simulink model "x35BusNetworkElectricityTransmissionModel"  (R2023b)
settings: Solver=VariableStepAuto  StartTime=0.0  StopTime=0.8  RelTol=1e-3
model workspace (MAT data in the model file):
  Compensation_Ki = 30
  Compensation_Kp = 3
  DC_Ki = 400
  DC_Kp = 8
  F = 0.01
  Flux_min = 0.5
  Grid_Freq_PWM = 2700
  Grid_Ireg_Ki = 5
  Grid_Ireg_Kp = 0.83
  Grid_Ireg_lim = 1.1
  Grid_Modindex_Upper = 1.1
  Grid_conv_Imax = 0.8
  H = 0.685
  Idref_max = 0.9
  Iqref_Tc = 0.3
  Ki_Var = 0.05
  Ki_Vreg = 20
  Ksh = 1.1
  L_pu = 0.3
  Llr = 0.16
  Lls = 0.18
  Lm = 2.9
  Nb_wt = 6
  P_mech = 1080000
  Pitch_Ki = 0
  Pitch_Kp = 150
  Pitch_Max = 27
  Pitch_Tc = 0.01
  Pitch_rate = 10
  Q_Filt = 50
  R_pu = 0.003
  Rotor_Freq_PWM = 1620
  Rotor_Ireg_Ki = 8
  Rotor_Ireg_Kp = 0.6
  Rotor_Ireg_lim = 0.1
  Rotor_Modindex_Upper = 2
  Rr = 0.016
  Rs = 0.023
  T_set = 0.0001
  Tp = 5e-05
  Ts = 5e-06
  Var_C_Filt = 720000
  Var_reg_max = 1.1
  Var_reg_min = 0.9
  WT_Coeff = [0.645 116 0.4 5 21 0.00912 0.08 0.035]
  WT_H = 4.32
  WT_IGBTRon = 5.931
  WT_Param = [91.204 10143]
  Wind_Freq_Filt = 10000
  Wind_Freq_nom = 60
  Wind_P_nom = 1200000
  Wind_Rotor_V_nom = 1950
  Wind_V_nom = 500
  Zeta_Filt = 0.707106781187
  init = [-0.2 0 0 0 0 0 0 0]
  p = 3
  torque0 = 0.83
  v_Ki = 0.1
  v_Kp = 3.6
  v_Max = 1.2
  v_Min = 0.7
  v_T = 5
  vreg_max = 1
  wind_VDC_nom = 1150
  wt0 = 1.2
undefined symbols (not defined in the file): D1, D11, Delta, DiscIntNeverNeededParam, Ion, Lithium, P, Q
libraries: powerlib_extras x144, spsSeriesRLCBranchLib x67, spsLoadFlowBusLib x43, spsThreePhaseTransformerTwoWindingsLib x32, spsThreePhaseSeriesRLCLoadLib x31, spsThreePhaseVIMeasurementLib x26, simulink_extras x26, spsDistributedParametersLineLib x22, spsGenericPowerSystemStabilizerLib x20, spsSynchronousMachinepuStandardLib x10, spsExcitationSystemLib x10, spsHydraulicTurbineandGovernorLib x10
(part 5 of 16)

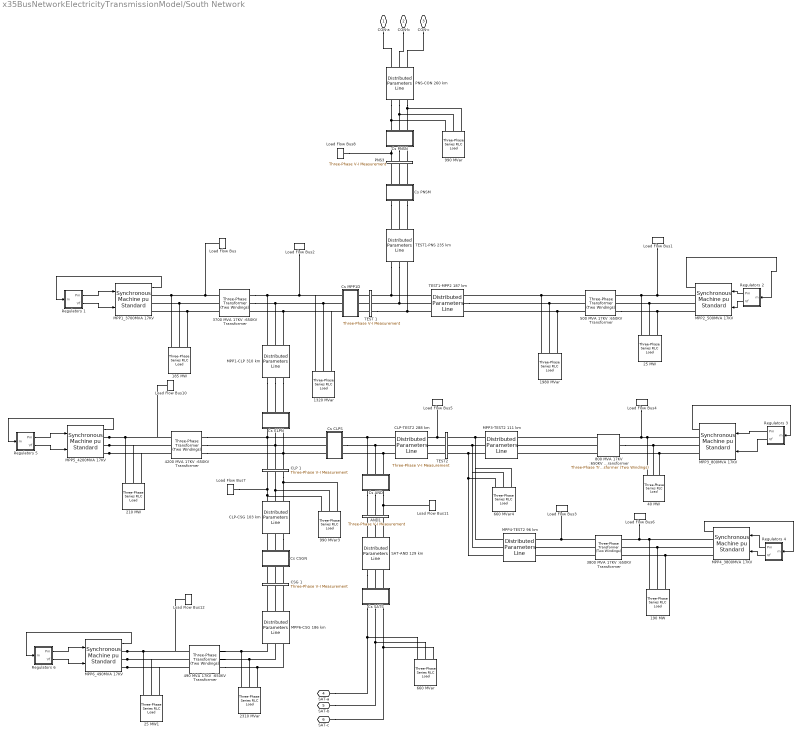
== system x35BusNetworkElectricityTransmissionModel/South Network ==
  " SAT-AND 129 km" : spsDistributedParametersLineLib/Distributed Parameters Line  Phases=3  Length=129  Frequency=60  Resistance=[0.01273 0.3864]/6  Inductance="[0.9337e-3  4.1264e-3]/6"  Capacitance=[12.74e-9 7.751e-9]*6  x1=[-0.00078 1.73015070651852e-08 -160788.800409401 -239334.964150814;-0.00072 1.8256737808598e-08 -155334.496074464 -242910.417917869;-0.00066 1.92026280676021e-08 -149800.719741084 -246361.594226648;-0.0006 2.01386939072632e-08 -144190.302591486 -249686.727391582;-0.00054 2.10644564190009e-08 -138506.115018751 -252884.116213103;-0.00048 2.19794419656084e-08 -132751.065158274 -255952.124848007;-0.00042 2.28831824235728e-08 -126928.097399904 -258889.183646388;-0.00036 2.37752154225767e-08 -121040.190881543 -261693.789954693;-0.0003 2.4655084582055e-08 -115090.357964961 -264364.508884513;-0.00024 2.55223397446875e-08 -109081.642694619 -266899.974046692;-0.00018 2.6376537206708e-08 -103017.119240278 -269298.888250405;-0.00012 2.72172399449112e-08 -96899.8903241954 -271560.024166817;-6e-05 2.80440178402418e-08 -90733.0856337191 -273682.224957013]  x2=[-0.00078 5.22592266110193e-08 -88973.713875581 -231973.83539445;-0.00072 5.48882545652481e-08 -83704.2752060405 -233926.888762085;-0.00066 5.7489200674223e-08 -78392.0118826275 -235760.260810956;-0.0006 6.00607342458547e-08 -73039.6417574174 -237473.013554048;-0.00054 6.26015396360514e-08 -67649.9032018668 -239064.27071541;-0.00048 6.51103169218269e-08 -62225.5537058117 -240533.218178473;-0.00042 6.75857825663648e-08 -56769.3684666847 -241879.104402573;-0.00036 7.00266700757002e-08 -51284.1389696728 -243101.240807449;-0.0003 7.24317306466807e-08 -45772.671559542 -244199.002125534;-0.00024 7.47997338058778e-08 -40237.7860048597 -245171.826721852;-0.00018 7.71294680391197e-08 -34682.3140553485 -246019.216881365;-0.00012 7.94197414113241e-08 -29109.0979931111 -246740.739063609;-6e-05 8.16693821763144e-08 -23520.9891784661 -247336.024124503]  x3=[-0.00078 -1.72880421705233e-09 -2677.59154686044 -14439.5075300877;-0.00072 -1.68724420508278e-09 -2350.32071608935 -14496.375500878;-0.00066 -1.64482096780123e-09 -2021.84741781098 -14545.8268580998;-0.0006 -1.60155620971975e-09 -1692.33970503421 -14587.8363015251;-0.00054 -1.55747206588802e-09 -1361.96615999351 -14622.3823383462;-0.00048 -1.51259109056861e-09 -1030.89580789911 -14649.4472941725;-0.00042 -1.4669362456978e-09 -699.298030460621 -14669.0173220725;-0.00036 -1.42053088913782e-09 -367.34247922821 -14681.0824096582;-0.0003 -1.37339876272656e-09 -35.1989887957174 -14685.6363842078;-0.00024 -1.32556398013081e-09 296.962510089846 -14682.676915824;-0.00018 -1.27705101450921e-09 628.972077468011 -14672.2055186254;-0.00012 -1.2278846859914e-09 960.659851109276 -14654.2275499722;-6e-05 -1.17809014897953e-09 1291.85613341976 -14628.7522077255]  x4=[-0.00078 2.10158311278446e-09 -3708.19041372056 4505.23785529734;-0.00072 2.08978742581233e-09 -3809.13872188143 4420.21514552939;-0.00066 2.07692256497832e-09 -3908.1382042874 4332.93097201679;-0.0006 2.06299511218296e-09 -4005.13821097396 4243.42999095556;-0.00054 2.04801219296843e-09 -4100.08911494535 4151.75799270137;-0.00048 2.03198147287307e-09 -4192.94233756459 4057.96187834246;-0.00042 2.01491115350949e-09 -4283.65037340727 3962.08963570407;-0.00036 1.99680996836849e-09 -4372.16681456616 3864.19031479706;-0.0003 1.97768717835087e-09 -4458.44637439435 3764.31400272297;-0.00024 1.95755256702935e-09 -4542.4449106748 3662.51179804856;-0.00018 1.93641643564312e-09 -4624.11944820421 3558.83578466283;-0.00012 1.91428959782756e-09 -4703.42820078001 3453.33900512995;-6e-05 1.89118337408174e-09 -4780.33059257894 3346.07543355167]  x5=0.000729548621424508  V1=[2.188e-18 3.182e-07 3.182e-07;377 377 377;0.6306 1.295 -0.2758]  V2=[1.209e-19 1.011e-07 1.011e-07;377 377 377;-2.255 -1.798 2.915]  I1=[1.016e-20 9.164e-09 9.164e-09;377 377 377;2.19 2.786 1.215]  I2=[1.089e-20 9.22e-09 9.22e-09;377 377 377;-0.7019 -0.2685 -1.839]  nHarmo=1  Measurements=None  Decoupling=off  VsMag0=0  VrMag0=0  VsAngle0=0  VrAngle0=0  IsMag0=0  IrMag0=0  IsAngle0=0  IrAngle0=0
      settings: LibrarySourceBlock=sps_lib/Power Grid Elements/Distributed Parameters Line
  1320 MVar : spsThreePhaseSeriesRLCLoadLib/Three-Phase Series RLC Load  LConnTagsString=A|B|C  Configuration=Y (grounded)  NominalVoltage=650e3  Vabc=[1e3 1e3 1e3]  Vabcp=[1e3 1e3 1e3]  NominalFrequency=60  UnbalancedPower=off  ActivePower=4400e3  InductivePower=1320e6  CapacitivePower=0  Pabc=[10e3 9e3 11e3]  QLabc=[100 90 110]  QCabc=[100 90 110]  Pabcp=[10e3 9e3 11e3]  QLabcp=[100 90 110]  QCabcp=[100 90 110]  Measurements=None  LoadType=constant Z
  185 MW : spsThreePhaseSeriesRLCLoadLib/Three-Phase Series RLC Load  LConnTagsString=A|B|C  Configuration=Y (grounded)  NominalVoltage=17e3  Vabc=[1e3 1e3 1e3]  Vabcp=[1e3 1e3 1e3]  NominalFrequency=60  UnbalancedPower=off  ActivePower=185e6  InductivePower=0  CapacitivePower=0  Pabc=[10e3 9e3 11e3]  QLabc=[100 90 110]  QCabc=[100 90 110]  Pabcp=[10e3 9e3 11e3]  QLabcp=[100 90 110]  QCabcp=[100 90 110]  Measurements=None  LoadType=constant Z
  190 MW : spsThreePhaseSeriesRLCLoadLib/Three-Phase Series RLC Load  LConnTagsString=A|B|C  Configuration=Y (grounded)  NominalVoltage=17e3  Vabc=[1e3 1e3 1e3]  Vabcp=[1e3 1e3 1e3]  NominalFrequency=60  UnbalancedPower=off  ActivePower=190e6  InductivePower=0  CapacitivePower=0  Pabc=[10e3 9e3 11e3]  QLabc=[100 90 110]  QCabc=[100 90 110]  Pabcp=[10e3 9e3 11e3]  QLabcp=[100 90 110]  QCabcp=[100 90 110]  Measurements=None  LoadType=constant Z
  1980 MVar : spsThreePhaseSeriesRLCLoadLib/Three-Phase Series RLC Load  LConnTagsString=A|B|C  Configuration=Y (grounded)  NominalVoltage=650e3  Vabc=[1e3 1e3 1e3]  Vabcp=[1e3 1e3 1e3]  NominalFrequency=60  UnbalancedPower=off  ActivePower=4400e3  InductivePower=1320e6  CapacitivePower=0  Pabc=[10e3 9e3 11e3]  QLabc=[100 90 110]  QCabc=[100 90 110]  Pabcp=[10e3 9e3 11e3]  QLabcp=[100 90 110]  QCabcp=[100 90 110]  Measurements=None  LoadType=constant Z
  210 MW : spsThreePhaseSeriesRLCLoadLib/Three-Phase Series RLC Load  LConnTagsString=A|B|C  Configuration=Y (grounded)  NominalVoltage=17e3  Vabc=[1e3 1e3 1e3]  Vabcp=[1e3 1e3 1e3]  NominalFrequency=60  UnbalancedPower=off  ActivePower=210e6  InductivePower=0  CapacitivePower=0  Pabc=[10e3 9e3 11e3]  QLabc=[100 90 110]  QCabc=[100 90 110]  Pabcp=[10e3 9e3 11e3]  QLabcp=[100 90 110]  QCabcp=[100 90 110]  Measurements=None  LoadType=constant Z
  2310 MVar : spsThreePhaseSeriesRLCLoadLib/Three-Phase Series RLC Load  LConnTagsString=A|B|C  Configuration=Y (grounded)  NominalVoltage=650e3  Vabc=[1e3 1e3 1e3]  Vabcp=[1e3 1e3 1e3]  NominalFrequency=60  UnbalancedPower=off  ActivePower=7700e3  InductivePower=2310e6  CapacitivePower=0  Pabc=[10e3 9e3 11e3]  QLabc=[100 90 110]  QCabc=[100 90 110]  Pabcp=[10e3 9e3 11e3]  QLabcp=[100 90 110]  QCabcp=[100 90 110]  Measurements=None  LoadType=constant Z
  25 MW : spsThreePhaseSeriesRLCLoadLib/Three-Phase Series RLC Load  LConnTagsString=A|B|C  Configuration=Y (grounded)  NominalVoltage=17e3  Vabc=[1e3 1e3 1e3]  Vabcp=[1e3 1e3 1e3]  NominalFrequency=60  UnbalancedPower=off  ActivePower=25e6  InductivePower=0  CapacitivePower=0  Pabc=[10e3 9e3 11e3]  QLabc=[100 90 110]  QCabc=[100 90 110]  Pabcp=[10e3 9e3 11e3]  QLabcp=[100 90 110]  QCabcp=[100 90 110]  Measurements=None  LoadType=constant Z
  25 MW1 : spsThreePhaseSeriesRLCLoadLib/Three-Phase Series RLC Load  LConnTagsString=A|B|C  Configuration=Y (grounded)  NominalVoltage=17e3  Vabc=[1e3 1e3 1e3]  Vabcp=[1e3 1e3 1e3]  NominalFrequency=60  UnbalancedPower=off  ActivePower=25e6  InductivePower=0  CapacitivePower=0  Pabc=[10e3 9e3 11e3]  QLabc=[100 90 110]  QCabc=[100 90 110]  Pabcp=[10e3 9e3 11e3]  QLabcp=[100 90 110]  QCabcp=[100 90 110]  Measurements=None  LoadType=constant Z
  "3700 MVA 17KV :650KV Transformer " : spsThreePhaseTransformerTwoWindingsLib/Three-Phase Transformer (Two Windings)  Winding1Connection=Delta (D1)  Winding2Connection=Yg  CoreType=Three single-phase transformers  SetSaturation=off  Hysteresis=off  DataFile='hysteresis'  SetInitialFlux=off  Measurements=None  UNITS=pu  NominalPower=[ 3700e6 , 60 ]  Winding1=[ 17e3 , 0.002 , 0.08 ]  Winding2=[ 650e3 , 0.002 , 0.08 ]  Rm=500  Lm=500  L0=0.5  Saturation=[ 0,0 ; 0.0024,1.2 ; 1.0,1.52 ]  InitialFluxes=[ 0.8 , -0.8 , 0.7 ]  BreakLoop=off  DiscreteSolver=Trapezoidal iterative  DataType=off  TransfoNumber=1
  3800 MVA 17KV :650KV Transformer : spsThreePhaseTransformerTwoWindingsLib/Three-Phase Transformer (Two Windings)  Winding1Connection=Yg  Winding2Connection=Delta (D1)  CoreType=Three single-phase transformers  SetSaturation=off  Hysteresis=off  DataFile='hysteresis'  SetInitialFlux=off  Measurements=None  UNITS=pu  NominalPower=[ 3800e6 , 60 ]  Winding1=[ 650e3 , 0.002 , 0.08 ]  Winding2=[ 17e3 , 0.002 , 0.08 ]  Rm=500  Lm=500  L0=0.5  Saturation=[ 0,0 ; 0.0024,1.2 ; 1.0,1.52 ]  InitialFluxes=[ 0.8 , -0.8 , 0.7 ]  BreakLoop=off  DiscreteSolver=Trapezoidal iterative  DataType=off  TransfoNumber=1
  40 MW : spsThreePhaseSeriesRLCLoadLib/Three-Phase Series RLC Load  LConnTagsString=A|B|C  Configuration=Y (grounded)  NominalVoltage=17e3  Vabc=[1e3 1e3 1e3]  Vabcp=[1e3 1e3 1e3]  NominalFrequency=60  UnbalancedPower=off  ActivePower=40e6  InductivePower=0  CapacitivePower=0  Pabc=[10e3 9e3 11e3]  QLabc=[100 90 110]  QCabc=[100 90 110]  Pabcp=[10e3 9e3 11e3]  QLabcp=[100 90 110]  QCabcp=[100 90 110]  Measurements=None  LoadType=constant Z
  4200 MVA 17KV :650KV Transformer : spsThreePhaseTransformerTwoWindingsLib/Three-Phase Transformer (Two Windings)  Winding1Connection=Delta (D1)  Winding2Connection=Yg  CoreType=Three single-phase transformers  SetSaturation=off  Hysteresis=off  DataFile='hysteresis'  SetInitialFlux=off  Measurements=None  UNITS=pu  NominalPower=[ 4200e6 , 60 ]  Winding1=[ 17e3 , 0.002 , 0.08 ]  Winding2=[ 650e3 , 0.002 , 0.08 ]  Rm=500  Lm=500  L0=0.5  Saturation=[ 0,0 ; 0.0024,1.2 ; 1.0,1.52 ]  InitialFluxes=[ 0.8 , -0.8 , 0.7 ]  BreakLoop=off  DiscreteSolver=Trapezoidal iterative  DataType=off  TransfoNumber=1
  490 MVA 17KV :650KV Transformer : spsThreePhaseTransformerTwoWindingsLib/Three-Phase Transformer (Two Windings)  Winding1Connection=Delta (D1)  Winding2Connection=Yg  CoreType=Three single-phase transformers  SetSaturation=off  Hysteresis=off  DataFile='hysteresis'  SetInitialFlux=off  Measurements=None  UNITS=pu  NominalPower=[ 490e6 , 60 ]  Winding1=[ 17e3 , 0.002 , 0.08 ]  Winding2=[ 650e3 , 0.002 , 0.08 ]  Rm=500  Lm=500  L0=0.5  Saturation=[ 0,0 ; 0.0024,1.2 ; 1.0,1.52 ]  InitialFluxes=[ 0.8 , -0.8 , 0.7 ]  BreakLoop=off  DiscreteSolver=Trapezoidal iterative  DataType=off  TransfoNumber=1
  "500 MVA 17KV :650KV Transformer " : spsThreePhaseTransformerTwoWindingsLib/Three-Phase Transformer (Two Windings)  Winding1Connection=Yg  Winding2Connection=Delta (D1)  CoreType=Three single-phase transformers  SetSaturation=off  Hysteresis=off  DataFile='hysteresis'  SetInitialFlux=off  Measurements=None  UNITS=pu  NominalPower=[ 500e6 , 60 ]  Winding1=[650e3 , 0.002 , 0.08 ]  Winding2=[17e3 , 0.002 , 0.08 ]  Rm=500  Lm=500  L0=0.5  Saturation=[ 0,0 ; 0.0024,1.2 ; 1.0,1.52 ]  InitialFluxes=[ 0.8 , -0.8 , 0.7 ]  BreakLoop=off  DiscreteSolver=Trapezoidal iterative  DataType=off  TransfoNumber=1
  660 MVar : spsThreePhaseSeriesRLCLoadLib/Three-Phase Series RLC Load  LConnTagsString=A|B|C  Configuration=Y (grounded)  NominalVoltage=650e3  Vabc=[1e3 1e3 1e3]  Vabcp=[1e3 1e3 1e3]  NominalFrequency=60  UnbalancedPower=off  ActivePower=2200e3  InductivePower=660e6  CapacitivePower=0  Pabc=[10e3 9e3 11e3]  QLabc=[100 90 110]  QCabc=[100 90 110]  Pabcp=[10e3 9e3 11e3]  QLabcp=[100 90 110]  QCabcp=[100 90 110]  Measurements=None  LoadType=constant Z
  660 MVar4 : spsThreePhaseSeriesRLCLoadLib/Three-Phase Series RLC Load  LConnTagsString=A|B|C  Configuration=Y (grounded)  NominalVoltage=650e3  Vabc=[1e3 1e3 1e3]  Vabcp=[1e3 1e3 1e3]  NominalFrequency=60  UnbalancedPower=off  ActivePower=2200e3  InductivePower=660e6  CapacitivePower=0  Pabc=[10e3 9e3 11e3]  QLabc=[100 90 110]  QCabc=[100 90 110]  Pabcp=[10e3 9e3 11e3]  QLabcp=[100 90 110]  QCabcp=[100 90 110]  Measurements=None  LoadType=constant Z
  800 MVA 17KV :650KV Transformer : spsThreePhaseTransformerTwoWindingsLib/Three-Phase Transformer (Two Windings)  Winding1Connection=Yg  Winding2Connection=Delta (D1)  CoreType=Three single-phase transformers  SetSaturation=off  Hysteresis=off  DataFile='hysteresis'  SetInitialFlux=off  Measurements=None  UNITS=pu  NominalPower=[ 800e6 , 60 ]  Winding1=[650e3 , 0.002 , 0.08 ]  Winding2=[ 17e3 , 0.002 , 0.08 ]  Rm=500  Lm=500  L0=0.5  Saturation=[ 0,0 ; 0.0024,1.2 ; 1.0,1.52 ]  InitialFluxes=[ 0.8 , -0.8 , 0.7 ]  BreakLoop=off  DiscreteSolver=Trapezoidal iterative  DataType=off  TransfoNumber=1
  990 MVar : spsThreePhaseSeriesRLCLoadLib/Three-Phase Series RLC Load  LConnTagsString=A|B|C  Configuration=Y (grounded)  NominalVoltage=650e3  Vabc=[1e3 1e3 1e3]  Vabcp=[1e3 1e3 1e3]  NominalFrequency=60  UnbalancedPower=off  ActivePower=2200e3  InductivePower=660e6  CapacitivePower=0  Pabc=[10e3 9e3 11e3]  QLabc=[100 90 110]  QCabc=[100 90 110]  Pabcp=[10e3 9e3 11e3]  QLabcp=[100 90 110]  QCabcp=[100 90 110]  Measurements=None  LoadType=constant Z
  990 MVar3 : spsThreePhaseSeriesRLCLoadLib/Three-Phase Series RLC Load  LConnTagsString=A|B|C  Configuration=Y (grounded)  NominalVoltage=650e3  Vabc=[1e3 1e3 1e3]  Vabcp=[1e3 1e3 1e3]  NominalFrequency=60  UnbalancedPower=off  ActivePower=3300e3  InductivePower=990e6  CapacitivePower=0  Pabc=[10e3 9e3 11e3]  QLabc=[100 90 110]  QCabc=[100 90 110]  Pabcp=[10e3 9e3 11e3]  QLabcp=[100 90 110]  QCabcp=[100 90 110]  Measurements=None  LoadType=constant Z
  AND1 : spsThreePhaseVIMeasurementLib/Three-Phase V-I Measurement  VoltageMeasurement=no  SetLabelV=off  LabelV=Vabc  Vpu=off  VpuLL=off  CurrentMeasurement=no  SetLabelI=off  LabelI=Iabc  Ipu=off  Pbase=100e6  Vbase=500e3  OutputType=Complex  PhasorSimulation=off  PSBequivalent=0
  CLP 1 : spsThreePhaseVIMeasurementLib/Three-Phase V-I Measurement  VoltageMeasurement=no  SetLabelV=off  LabelV=Vabc  Vpu=off  VpuLL=off  CurrentMeasurement=no  SetLabelI=off  LabelI=Iabc  Ipu=off  Pbase=100e6  Vbase=500e3  OutputType=Complex  PhasorSimulation=off  PSBequivalent=0
  CLP-CSG 103 km : spsDistributedParametersLineLib/Distributed Parameters Line  Phases=3  Length=103  Frequency=60  Resistance=[0.01273 0.3864]/6  Inductance="[0.9337e-3  4.1264e-3]/6"  Capacitance=[12.74e-9 7.751e-9]*6  x1=[-0.0006 3.92711037156733e-08 -150312.081292197 -256752.693722347;-0.00054 4.02003694351059e-08 -144466.512887676 -260086.735304661;-0.00048 4.1109067902718e-08 -138547.032745726 -263287.711707343;-0.00042 4.19967342115829e-08 -132556.669381769 -266353.985251718;-0.00036 4.28629142152147e-08 -126498.487576391 -269283.987175583;-0.0003 4.37071647599184e-08 -120375.586807346 -272076.218435812;-0.00024 4.45290539115154e-08 -114191.099663804 -274729.250475299;-0.00018 4.53281611763289e-08 -107948.190243666 -277241.72595383;-0.00012 4.61040777163166e-08 -101650.052534746 -279612.359442526;-6e-05 4.68564065582391e-08 -95299.908780672 -281839.938081488]  x2=[-0.0006 3.46834464690486e-08 -152766.904511302 -257465.980570063;-0.00054 3.58237170617729e-08 -146904.575209073 -260855.361892625;-0.00048 3.69456595789022e-08 -140967.086811682 -264111.28479199;-0.00042 3.80487000139136e-08 -134957.477047906 -267232.08347784;-0.00036 3.91322740309387e-08 -128878.820545144 -270216.161291901;-0.0003 4.01958272534884e-08 -122734.227256386 -273061.991524825;-0.00024 4.12388155480817e-08 -116526.840869094 -275768.118197279;-0.00018 4.22607053026349e-08 -110259.837196846 -278333.156804855;-0.00012 4.32609736994672e-08 -103936.422554521 -280755.795026404;-6e-05 4.42391089827839e-08 -97559.8321178918 -283034.793395447]  x3=[-0.0006 -8.57836265093248e-11 -3832.5749236527 -5045.22121215062;-0.00054 -7.93836822522111e-11 -3717.48388598462 -5130.61468863092;-0.00048 -7.29431238364154e-11 -3600.49091486927 -5213.38324783366;-0.00042 -6.6465246370631e-11 -3481.65586607244 -5293.48454383456;-0.00036 -5.99533640566669e-11 -3361.03953780094 -5370.87759533049;-0.0003 -5.34108084938405e-11 -3238.70363959702 -5445.52280660624;-0.00024 -4.68409269744705e-11 -3114.71076076672 -5517.38198779243;-0.00018 -4.02470807713395e-11 -2989.12433835798 -5586.41837440418;-0.00012 -3.36326434180053e-11 -2862.00862470507 -5652.59664615044;-6e-05 -2.70009989828387e-11 -2733.42865455591 -5715.88294500454]  x4=[-0.0006 5.88767514656271e-10 -3622.67392283929 -5860.74468145355;-0.00054 6.00102975589294e-10 -3489.19149359268 -5941.18214271376;-0.00048 6.11131412751377e-10 -3353.92392950511 -6018.57998540933;-0.00042 6.21847183790286e-10 -3216.94043596181 -6092.89861137379;-0.00036 6.32244806319553e-10 -3078.31109624924 -6164.09999782485;-0.0003 6.42318960723366e-10 -2938.10683569919 -6232.14771681756;-0.00024 6.52064492878184e-10 -2796.39938540202 -6297.00695388149;-0.00018 6.61476416789678e-10 -2653.26124550776 -6358.6445258325;-0.00012 6.70549917143664e-10 -2508.76564813367 -6417.02889774986;-6e-05 6.79280351769702e-10 -2362.98651989733 -6472.13019911006]  x5=0.000582507814005615  V1=[1.056e-22 6.221e-12 6.221e-12;377 377 377;0.3647 1.373 -0.1974]  V2=[1.588e-22 9.824e-12 9.824e-12;377 377 377;0.3755 1.375 -0.1957]  I1=[3.913e-25 1.044e-13 1.044e-13;377 377 377;-0.5956 0.0636 -1.507]  I2=[3.097e-25 1.021e-13 1.021e-13;377 377 377;1.525 2.624 1.053]  nHarmo=1  Measurements=None  Decoupling=off  VsMag0=0  VrMag0=0  VsAngle0=0  VrAngle0=0  IsMag0=0  IrMag0=0  IsAngle0=0  IrAngle0=0
      settings: LibrarySourceBlock=sps_lib/Power Grid Elements/Distributed Parameters Line
  CLP-TEST2 288 km : spsDistributedParametersLineLib/Distributed Parameters Line  Phases=3  Length=288  Frequency=60  Resistance=[0.01273 0.3864]/6  Inductance="[0.9337e-3  4.1264e-3]/6"  Capacitance=[12.74e-9 7.751e-9]*6  x1=[-0.00168 -5.65553918327e-09 0 0;-0.00162 -5.14288112742245e-09 0 0;-0.00156 -4.6275918785606e-09 0 0;-0.0015 -4.10993506818561e-09 0 0;-0.00144 -3.59017553908687e-09 0 0;-0.00138 -3.06857920984352e-09 0 0;-0.00132 -2.54541293877558e-09 0 0;-0.00126 -2.02094438741434e-09 0 0;-0.0012 -1.49544188356175e-09 0 0;-0.00114 -9.69174284008934e-10 0 0;-0.00108 -4.42410836984137e-10 0 0;-0.00102 8.457895559967e-11 -80544.0337060146 -208122.10077131;-0.00096 6.11525476026955e-10 -75816.2183893697 -209890.593985758;-0.0009 1.13815912872101e-09 -71049.6140944741 -211551.70329399;-0.00084 1.66421047817406e-09 -66246.6595041619 -213104.578841792;-0.00078 2.18941038679539e-09 -61409.8118987498 -214548.426149338;-0.00072 2.71349015260719e-09 -56541.5458988475 -215882.506517667;-0.00066 3.23618164671738e-09 -51644.3521992956 -217106.137406612;-0.0006 3.75721745049934e-09 -46720.7362948807 -218218.692783999;-0.00054 4.27633099240824e-09 -41773.2171984774 -219219.60344594;-0.00048 4.79325668436391e-09 -36804.326152275 -220108.357308046;-0.00042 5.30773005763066e-09 -31816.6053327474 -220884.499667418;-0.00036 5.81948789812434e-09 -26812.6065500283 -221547.633435284;-0.0003 6.32826838107758e-09 -21794.8899423582 -222097.419340155;-0.00024 6.8338112049941e-09 -16766.0226662703 -222533.576101403;-0.00018 7.33585772482384e-09 -11728.5775831858 -222855.880573169;-0.00012 7.83415108429049e-09 -6685.13194309062 -223064.167858532;-6e-05 8.32843634730394e-09 -1638.26606596631 -223158.331393866]  x2=[-0.00168 4.10808268888269e-08 0 0;-0.00162 4.02895288423073e-08 0 0;-0.00156 3.94776179283671e-08 0 0;-0.0015 3.86455095356323e-08 0 0;-0.00144 3.77936293861321e-08 0 0;-0.00138 3.6922413317492e-08 0 0;-0.00132 3.6032307059951e-08 0 0;-0.00126 3.51237660083175e-08 0 0;-0.0012 3.41972549889817e-08 0 0;-0.00114 3.32532480221008e-08 0 0;-0.00108 3.22922280790825e-08 0 0;-0.00102 3.13146868354871e-08 -161682.012206487 -227631.966150118;-0.00096 3.03211244194778e-08 -156492.170905739 -231230.614921688;-0.0009 2.93120491559456e-08 -151222.265318713 -234710.961838014;-0.00084 2.82879773064408e-08 -145874.991626483 -238071.226289303;-0.00078 2.72494328050443e-08 -140453.085593078 -241309.689102173;-0.00072 2.61969469903131e-08 -134959.321165808 -244424.693419207;-0.00066 2.51310583334377e-08 -129396.509056068 -247414.645546639;-0.0006 2.40523121627504e-08 -123767.495301323 -250278.015769713;-0.00054 2.2961260384725e-08 -118075.159809021 -253013.339135312;-0.00048 2.18584612016114e-08 -112322.414883183 -255619.216201462;-0.00042 2.07444788258492e-08 -106512.203734411 -258094.313753302;-0.00036 1.96198831914058e-08 -100647.498974089 -260437.365485191;-0.0003 1.84852496621879e-08 -94731.3010935404 -262647.17264857;-0.00024 1.73411587376747e-08 -88766.6369289189 -264722.604665259;-0.00018 1.61881957559235e-08 -82756.5581126257 -266662.59970589;-0.00012 1.50269505941001e-08 -76704.1395120367 -268466.165233154;-6e-05 1.38580173666867e-08 -70612.4776563437 -270132.3785096]  x3=[-0.00168 7.52518123679813e-10 0 0;-0.00162 7.65283733086246e-10 0 0;-0.00156 7.77657809194014e-10 0 0;-0.0015 7.89634021197134e-10 0 0;-0.00144 8.0120624184425e-10 0 0;-0.00138 8.12368550573451e-10 0 0;-0.00132 8.23115236541332e-10 0 0;-0.00126 8.33440801544778e-10 0 0;-0.0012 8.43339962833939e-10 0 0;-0.00114 8.52807655814983e-10 0 0;-0.00108 8.61839036641239e-10 0 0;-0.00102 8.70429484691394e-10 -3978.72203483737 606.251412650929;-0.00096 8.78574604933493e-10 -3991.41569883362 516.107179639946;-0.0009 8.86270230173517e-10 -4002.06728080546 425.698896659295;-0.00084 8.93512423187393e-10 -4010.67133120673 335.072818257102;-0.00078 9.00297478735355e-10 -4017.22344804628 244.275310409655;-0.00072 9.06621925457611e-10 -4021.72027914005 153.352826799713;-0.00066 9.12482527650356e-10 -4024.15952382617 62.3518850499466;-0.0006 9.17876286921216e-10 -4024.53993414198 -28.6809570763421;-0.00054 9.22800443723284e-10 -4022.86131546254 -119.699125495027;-0.00048 9.27252478766952e-10 -4019.12452660017 -210.656053629324;-0.00042 9.31230114308826e-10 -4013.33147936511 -301.505206234107;-0.00036 9.34731315317066e-10 -4005.48513758737 -392.200103204206;-0.0003 9.37754290512541e-10 -3995.58951560039 -482.69434335448;-0.00024 9.40297493285283e-10 -3983.64967618722 -572.941628159528;-0.00018 9.4235962248576e-10 -3969.67172799033 -662.895785440866;-0.00012 9.43939623090569e-10 -3953.66282238629 -752.510792989467;-6e-05 9.45036686742207e-10 -3935.63114982704 -841.740802111573]  x4=[-0.00168 -4.65200455930411e-10 0 0;-0.00162 -4.78156789174548e-10 0 0;-0.00156 -4.90868488570023e-10 0 0;-0.0015 -5.03329050576538e-10 0 0;-0.00144 -5.15532100140327e-10 0 0;-0.00138 -5.27471393955746e-10 0 0;-0.00132 -5.39140823659467e-10 0 0;-0.00126 -5.50534418955626e-10 0 0;-0.0012 -5.61646350670342e-10 0 0;-0.00114 -5.72470933734023e-10 0 0;-0.00108 -5.83002630089959e-10 0 0;-0.00102 -5.93236051527691e-10 -3152.23324771321 -9155.02576483706;-0.00096 -6.03165962439719e-10 -2944.36276871944 -9223.98050174141;-0.0009 -6.12787282500139e-10 -2734.98589932763 -9288.21607978152;-0.00084 -6.22095089263823e-10 -2524.20976061299 -9347.6996348487;-0.00078 -6.31084620684845e-10 -2312.14218954279 -9402.40073405707;-0.00072 -6.39751277552821e-10 -2098.89168380494 -9452.2913913135;-0.00066 -6.48090625845957e-10 -1884.5673462986 -9497.34608163588;-0.0006 -6.56098398999573e-10 -1669.27882931509 -9537.54175421211;-0.00054 -6.63770500088955e-10 -1453.13627843778 -9572.85784419338;-0.00048 -6.71103003925424e-10 -1236.25027618955 -9603.27628321548;-0.00042 -6.78092159064526e-10 -1018.73178545674 -9628.78150864295;-0.00036 -6.84734389725349e-10 -800.692092718491 -9649.36047153117;-0.0003 -6.91026297619951e-10 -582.242751110519 -9665.00264330247;-0.00024 -6.96964663691993e-10 -363.49552335247 -9675.70002113275;-0.00018 -7.02546449763664e-10 -144.562324568049 -9681.44713204583;-0.00012 -7.0776880009007e-10 74.4448349728254 -9682.24103571358;-6e-05 -7.12629042820287e-10 293.413907160545 -9678.08132596022]  x5=0.00162875971294774  V1=[1.245e-23 7.93e-13 7.93e-13;377 377 377;-1.837 -1.972 2.74]  V2=[6.065e-20 5.187e-08 5.187e-08;377 377 377;-2.594 -2.004 2.709]  I1=[1.297e-22 5.199e-10 5.199e-10;377 377 377;2.342 2.744 1.173]  I2=[1.117e-22 5.13e-10 5.13e-10;377 377 377;-1.44 -0.7735 -2.344]  nHarmo=1  Measurements=None  Decoupling=off  VsMag0=0  VrMag0=0  VsAngle0=0  VrAngle0=0  IsMag0=0  IrMag0=0  IsAngle0=0  IrAngle0=0
      settings: LibrarySourceBlock=sps_lib/Power Grid Elements/Distributed Parameters Line
  CSG 1 : spsThreePhaseVIMeasurementLib/Three-Phase V-I Measurement  VoltageMeasurement=no  SetLabelV=off  LabelV=Vabc  Vpu=off  VpuLL=off  CurrentMeasurement=no  SetLabelI=off  LabelI=Iabc  Ipu=off  Pbase=100e6  Vbase=500e3  OutputType=Complex  PhasorSimulation=off  PSBequivalent=0
  Cs AND : Subsystem
  Cs CLPN : Subsystem
  Cs CLPS : Subsystem
  Cs CSGN : Subsystem
  Cs MPP1D : Subsystem
  Cs PNSM : Subsystem
  Cs PNSN : Subsystem
  Cs SATS : Subsystem
  Load Flow Bus : spsLoadFlowBusLib/Load Flow Bus  LConnTagsString=a  Phases=single  Connectors=on one side  ID=BUS_1  Vbase=17e3  Vref=1  Vangle=0  VLF=1  VLFb=1  VLFc=1  angleLF=0  angleLFb=0  angleLFc=0
  Load Flow Bus1 : spsLoadFlowBusLib/Load Flow Bus  LConnTagsString=a  Phases=single  Connectors=on one side  ID=BUS_2  Vbase=17e3  Vref=1  Vangle=0  VLF=1  VLFb=1  VLFc=1  angleLF=0  angleLFb=0  angleLFc=0
  Load Flow Bus10 : spsLoadFlowBusLib/Load Flow Bus  LConnTagsString=a  Phases=single  Connectors=on one side  ID=BUS_5  Vbase=17e3  Vref=1  Vangle=0  VLF=1  VLFb=1  VLFc=1  angleLF=0  angleLFb=0  angleLFc=0
  Load Flow Bus11 : spsLoadFlowBusLib/Load Flow Bus  LConnTagsString=a  Phases=single  Connectors=on one side  ID=BUS_11  Vbase=650e3  Vref=1.031  Vangle=17.31  VLF=1  VLFb=1  VLFc=1  angleLF=0  angleLFb=0  angleLFc=0
  Load Flow Bus12 : spsLoadFlowBusLib/Load Flow Bus  LConnTagsString=a  Phases=single  Connectors=on one side  ID=BUS_6  Vbase=17e3  Vref=1  Vangle=0  VLF=1  VLFb=1  VLFc=1  angleLF=0  angleLFb=0  angleLFc=0
  Load Flow Bus2 : spsLoadFlowBusLib/Load Flow Bus  LConnTagsString=a  Phases=single  Connectors=on one side  ID=BUS_7  Vbase=650e3  Vref=1  Vangle=0  VLF=1  VLFb=1  VLFc=1  angleLF=0  angleLFb=0  angleLFc=0
  Load Flow Bus3 : spsLoadFlowBusLib/Load Flow Bus  LConnTagsString=a  Phases=single  Connectors=on one side  ID=BUS_9  Vbase=650e3  Vref=1.031  Vangle=17.31  VLF=1  VLFb=1  VLFc=1  angleLF=0  angleLFb=0  angleLFc=0
  Load Flow Bus4 : spsLoadFlowBusLib/Load Flow Bus  LConnTagsString=a  Phases=single  Connectors=on one side  ID=BUS_3  Vbase=17e3  Vref=1  Vangle=0  VLF=1  VLFb=1  VLFc=1  angleLF=0  angleLFb=0  angleLFc=0
  Load Flow Bus5 : spsLoadFlowBusLib/Load Flow Bus  LConnTagsString=a  Phases=single  Connectors=on one side  ID=BUS_8  Vbase=650e3  Vref=1.031  Vangle=17.31  VLF=1  VLFb=1  VLFc=1  angleLF=0  angleLFb=0  angleLFc=0
  Load Flow Bus6 : spsLoadFlowBusLib/Load Flow Bus  LConnTagsString=a  Phases=single  Connectors=on one side  ID=BUS_4  Vbase=17e3  Vref=1  Vangle=0  VLF=1  VLFb=1  VLFc=1  angleLF=0  angleLFb=0  angleLFc=0
  Load Flow Bus7 : spsLoadFlowBusLib/Load Flow Bus  LConnTagsString=a  Phases=single  Connectors=on one side  ID=BUS_10  Vbase=650e3  Vref=1.031  Vangle=17.31  VLF=1  VLFb=1  VLFc=1  angleLF=0  angleLFb=0  angleLFc=0
  Load Flow Bus8 : spsLoadFlowBusLib/Load Flow Bus  LConnTagsString=a  Phases=single  Connectors=on one side  ID=BUS_12  Vbase=650e3  Vref=1  Vangle=0  VLF=1  VLFb=1  VLFc=1  angleLF=0  angleLFb=0  angleLFc=0
  MPP1-CLP 310 km : spsDistributedParametersLineLib/Distributed Parameters Line  Phases=3  Length=310  Frequency=60  Resistance=[0.01273 0.3864]/6  Inductance="[0.9337e-3  4.1264e-3]/6"  Capacitance=[12.74e-9 7.751e-9]*6  x1=[-0.0018 -3.67236237919446e-09 -241463.12326215 -184949.845971911;-0.00174 -4.4351589562731e-09 -237218.227496092 -190363.864508858;-0.00168 -5.1956864240774e-09 -232851.966501558 -195680.489375202;-0.00162 -5.95355568270189e-09 -228366.574138352 -200897.000487421;-0.00156 -6.70837899223005e-09 -223764.345216088 -206010.728982042;-0.0015 -7.45977017110919e-09 -219047.634320121 -211019.058581075;-0.00144 -8.20734479372809e-09 -214218.854606902 -215919.426930554;-0.00138 -8.95072038709622e-09 -209280.476569356 -220709.326911483;-0.00132 -9.68951662652402e-09 -204235.026772939 -225386.307922525;-0.00126 -1.0423355530204e-08 -199085.086562995 -229947.977133773;-0.0012 -1.11518616525933e-08 -193833.290744096 -234392.00071097;-0.00114 -1.18746622764984e-08 -188482.326232025 -238716.105009536;-0.00108 -1.25913876037643e-08 -183034.930679101 -242918.077737814;-0.00102 -1.330167094447e-08 -177493.891073545 -246995.769088911;-0.00096 -1.40051489045339e-08 -171862.042313606 -250947.092840584;-0.0009 -1.47014615716329e-08 -166142.265757173 -254770.027422592;-0.00084 -1.539025269934e-08 -160337.487747623 -258462.616950961;-0.00078 -1.6071169889387e-08 -154450.678116646 -262022.972228658;-0.00072 -1.67438647719575e-08 -148484.848664823 -265449.271712135;-0.00066 -1.74079931839196e-08 -142443.051620739 -268739.762443265;-0.0006 -1.80632153449061e-08 -136328.378079401 -271892.76094619;-0.00054 -1.87091960311523e-08 -130143.956420778 -274906.654088614;-0.00048 -1.93456047470027e-08 -123892.950709267 -277779.899907115;-0.00042 -1.9972115893999e-08 -117578.559074895 -280511.028396042;-0.00036 -2.05884089374615e-08 -111204.012077098 -283098.642259593;-0.0003 -2.11941685704817e-08 -104772.571051908 -285541.417626702;-0.00024 -2.17890848752379e-08 -98287.5264433936 -287838.104728356;-0.00018 -2.2372853481556e-08 -91752.1961202061 -289987.528536993;-0.00012 -2.29451757226301e-08 -85169.9236780978 -291988.589367677;-6e-05 -2.35057587878264e-08 -78544.0767292766 -293840.263440713]  x2=[-0.0018 6.40456232512644e-08 -245614.223163535 -150961.63059626;-0.00174 6.49105874403913e-08 -242136.995633654 -156478.228205276;-0.00168 6.57423421735739e-08 -238535.886342629 -161914.768661358;-0.00162 6.65404619097217e-08 -234812.737684515 -167268.470529951;-0.00156 6.73045383160301e-08 -230969.454490961 -172536.594758255;-0.0015 6.80341804768912e-08 -227008.003056665 -177716.446076571;-0.00144 6.87290150938932e-08 -222930.410133379 -182805.374377252;-0.00138 6.9388686676807e-08 -218738.761892989 -187800.776070547;-0.00132 7.00128577254614e-08 -214435.202860187 -192700.095416644;-0.00126 7.06012089024145e-08 -210021.934815294 -197500.825833238;-0.0012 7.11534391963329e-08 -205501.215667791 -202200.51117794;-0.00114 7.1669266075994e-08 -200875.358301126 -206796.747004888;-0.00108 7.21484256348349e-08 -196146.729389405 -211287.181794903;-0.00102 7.25906727259714e-08 -191317.748186553 -215669.518158574;-0.00096 7.29957810876199e-08 -186390.885288583 -219941.514011641;-0.0009 7.33635434588569e-08 -181368.661369593 -224100.983722087;-0.00084 7.3693771685658e-08 -176253.645892137 -228145.799228351;-0.00078 7.39862968171604e-08 -171048.455792651 -232073.89112808;-0.00072 7.42409691921016e-08 -165755.754142569 -235883.249736875;-0.00066 7.44576585153887e-08 -160378.248785853 -239571.926116484;-0.0006 7.46362539247599e-08 -154918.69095361 -243138.033071911;-0.00054 7.47766640475039e-08 -149379.873856506 -246579.746116945;-0.00048 7.48788170472073e-08 -143764.631255714 -249895.304407595;-0.00042 7.49426606605078e-08 -138075.836013108 -253083.011642976;-0.00036 7.49681622238333e-08 -132316.398621448 -256141.236933164;-0.0003 7.49553086901128e-08 -126489.265715328 -259068.415633591;-0.00024 7.49041066354515e-08 -120597.418563615 -261863.050145546;-0.00018 7.48145822557667e-08 -114643.871544181 -264523.710682374;-0.00012 7.46867813533854e-08 -108631.67060169 -267049.03600098;-6e-05 7.45207693136106e-08 -102563.891689237 -269437.73409827]  x3=[-0.0018 -6.10415089722204e-10 -4228.04542535679 -2669.41799979454;-0.00174 -5.93830960446157e-10 -4166.58785836452 -2764.3636901512;-0.00168 -5.76943016278011e-10 -4102.99858803421 -2857.89508096441;-0.00162 -5.59759897402056e-10 -4037.31014781157 -2949.96431984637;-0.00156 -5.42290395019416e-10 -3969.55614511639 -3040.52430247322;-0.0015 -5.2454344685031e-10 -3899.77124414841 -3129.52869668449;-0.00144 -5.06528132561347e-10 -3827.99114815244 -3216.93196618751;-0.00138 -4.88253669120202e-10 -3754.25258115193 -3302.68939385455;-0.00132 -4.69729406080045e-10 -3678.59326916028 -3386.75710460101;-0.00126 -4.50964820796135e-10 -3601.05192087955 -3469.09208783268;-0.0012 -4.31969513577035e-10 -3521.66820789631 -3549.65221945077;-0.00114 -4.12753202772909e-10 -3440.48274438496 -3628.39628340335;-0.00108 -3.93325719803443e-10 -3357.53706632877 -3705.28399277229;-0.00102 -3.73697004127902e-10 -3272.87361026929 -3780.27601038475;-0.00096 -3.53877098159922e-10 -3186.53569159505 -3853.33396893883;-0.0009 -3.33876142129626e-10 -3098.56748238058 -3924.42049063298;-0.00084 -3.13704368895695e-10 -3009.01398878718 -3993.49920628916;-0.00078 -2.93372098710047e-10 -2917.92102803693 -4060.53477396002;-0.00072 -2.72889733937806e-10 -2825.33520497176 -4125.49289701047;-0.00066 -2.52267753735259e-10 -2731.30388820953 -4188.34034166447;-0.0006 -2.3151670868853e-10 -2635.8751859094 -4249.04495400804;-0.00054 -2.10647215415698e-10 -2539.09792115879 -4307.57567643982;-0.00048 -1.89669951135147e-10 -2441.02160699457 -4363.90256356068;-0.00042 -1.68595648202898e-10 -2341.69642107132 -4417.99679749438;-0.00036 -1.47435088621738e-10 -2241.17317998948 -4469.83070263128;-0.0003 -1.26199098524952e-10 -2139.50331329664 -4519.37775978774;-0.00024 -1.0489854263747e-10 -2036.73883717524 -4566.6126197738;-0.00018 -8.3544318717272e-11 -1932.93232783013 -4611.51111636228;-0.00012 -6.21473519798969e-11 -1828.13689458962 -4654.0502786527;-6e-05 -4.07185895088978e-11 -1722.40615273376 -4694.2083428236]  x4=[-0.0018 1.03524187542742e-09 -7958.21733101256 -2503.87978442016;-0.00174 1.02285847596155e-09 -7899.54929286735 -2683.23503240961;-0.00168 1.00995176319913e-09 -7836.83969933702 -2861.21748777599;-0.00162 9.9652834045289e-10 -7770.12063380835 -3037.7360914064;-0.00156 9.8259507539395e-10 -7699.42623098812 -3212.70053312154;-0.0015 9.68159096538169e-10 -7624.79265943907 -3386.02129788006;-0.00144 9.53227789599076e-10 -7546.25810307548 -3557.6097115761;-0.00138 9.37808793709199e-10 -7463.86274162754 -3727.37798640663;-0.00132 9.21909997511747e-10 -7377.64873008466 -3895.23926578529;-0.00126 9.05539535124629e-10 -7287.66017712819 -4061.10766877982;-0.0012 8.88705781978895e-10 -7193.94312256463 -4224.89833405037;-0.00114 8.71417350533706e-10 -7096.54551377077 -4386.52746326607;-0.00108 8.53683085870043e-10 -6995.51718116299 -4545.91236397785;-0.00102 8.35512061165399e-10 -6890.90981270303 -4702.97149192542;-0.00096 8.16913573051774e-10 -6782.77692745352 -4857.62449275681;-0.0009 7.97897136859349e-10 -6671.17384819661 -5009.79224313911;-0.00084 7.78472481748263e-10 -6556.15767312985 -5159.39689123951;-0.00078 7.58649545730997e-10 -6437.78724665365 -5306.36189655566;-0.00072 7.38438470587903e-10 -6316.12312926543 -5450.61206907523;-0.00066 7.17849596678483e-10 -6191.22756657574 -5592.07360774454;-0.0006 6.96893457651066e-10 -6063.16445746226 -5730.67413822648;-0.00054 6.75580775053604e-10 -5931.99932137794 -5866.34274992863;-0.00048 6.53922452848327e-10 -5797.79926483007 -5999.01003228236;-0.00042 6.31929571833076e-10 -5660.63294704729 -6128.60811025461;-0.00036 6.09613383972159e-10 -5520.57054485233 -6255.070679074;-0.0003 5.86985306639642e-10 -5377.68371675821 -6378.33303815356;-0.00024 5.64056916778006e-10 -5232.04556630643 -6498.33212419276;-0.00018 5.40839944975173e-10 -5083.73060466584 -6615.00654344184;-0.00012 5.17346269462918e-10 -4932.81471251136 -6728.29660311204;-6e-05 4.93587910039745e-10 -4779.37510120202 -6838.14434191546]  x5=0.0017531788576868  V1=[1.492e-21 4.488e-11 4.488e-11;377 377 377;2.889 -1.992 2.721]  V2=[1.003e-22 1.265e-11 1.265e-11;377 377 377;0.8549 1.122 -0.4483]  I1=[2.499e-24 5.251e-13 5.251e-13;377 377 377;-2.215 -0.7076 -2.278]  I2=[3.136e-24 5.274e-13 5.274e-13;377 377 377;1.561 2.663 1.092]  nHarmo=1  Measurements=None  Decoupling=off  VsMag0=0  VrMag0=0  VsAngle0=0  VrAngle0=0  IsMag0=0  IrMag0=0  IsAngle0=0  IrAngle0=0
      settings: LibrarySourceBlock=sps_lib/Power Grid Elements/Distributed Parameters Line
  MPP1_3700MVA 17KV : spsSynchronousMachinepuStandardLib/Synchronous Machine pu Standard  PresetModel=No  MechanicalLoad=Mechanical power Pm  ShowDetailedParameters=on  RotorType=Salient-pole  Units=per unit standard parameters  MeasurementBus=off  NominalParameters=[3700e6 17000 60]  Reactances1=[ 1.81, 0.3, 0.23, 1.76, 0.65, 0.25, 0.15 ]  Reactances2=[ 1.305, 0.296, 0.252, 0.474, 0.243, 0.18 ]  dAxisTimeConstants=Short-circuit  qAxisTimeConstants=Open-circuit  TimeConstants1="[ 4.4849  0.0681  0.1  ]"  TimeConstants2=[ 8.0, 0.03, 1.0, 0.07 ]  TimeConstants3="[  4.49  0.0681  0.0513  ]"  TimeConstants4=[ 8.0, 0.03, 0.3371, 0.0295 ]  TimeConstants5=[ 1.01, 0.053, 0.1 ]  TimeConstants6=[ 1.3201, 0.023, 1.0, 0.07 ]  TimeConstants7=[0.012 0.003 0.003]  TimeConstants8=[ 1.3201, 0.0231, 0.3371, 0.0295 ]  StatorResistance=2.8544e-3  Mechanical=[3.5 0 32]  PolePairs=20  InitialConditions=[0 -81.9543 0.907703 0.907703 0.907703 -8.76021 -128.76 111.24 1.25655]  SetSaturation=off  Saturation=[0.6404,0.7127,0.8441,0.9214,0.9956,1.082,1.19,1.316,1.457;0.7,0.7698,0.8872,0.9466,0.9969,1.046,1.1,1.151,1.201]  LoadFlowParameters=[1,0,0,0,0]  TsPowergui=0  TsBlock=-1  IterativeModel=Trapezoidal non iterative  IterativeDiscreteModel=Trapezoidal non iterative  BusType=PV  Pref=3000e6  Qref=0  Qmin=-inf  Qmax=inf  PLF=0  QLF=0
  MPP2_500MVA 17KV : spsSynchronousMachinepuStandardLib/Synchronous Machine pu Standard  PresetModel=No  MechanicalLoad=Mechanical power Pm  ShowDetailedParameters=on  RotorType=Salient-pole  Units=per unit standard parameters  MeasurementBus=off  NominalParameters=[500e6 17000 60]  Reactances1=[ 1.81, 0.3, 0.23, 1.76, 0.65, 0.25, 0.15 ]  Reactances2=[ 1.305, 0.296, 0.252, 0.474, 0.243, 0.18 ]  dAxisTimeConstants=Short-circuit  qAxisTimeConstants=Open-circuit  TimeConstants1="[ 4.4849  0.0681  0.1  ]"  TimeConstants2=[ 8.0, 0.03, 1.0, 0.07 ]  TimeConstants3="[  4.49  0.0681  0.0513  ]"  TimeConstants4=[ 8.0, 0.03, 0.3371, 0.0295 ]  TimeConstants5=[ 1.01, 0.053, 0.1 ]  TimeConstants6=[ 1.3201, 0.023, 1.0, 0.07 ]  TimeConstants7=[0.012 0.003 0.003]  TimeConstants8=[ 1.3201, 0.0231, 0.3371, 0.0295 ]  StatorResistance=2.8544e-3  Mechanical=[3.5 0 32]  PolePairs=20  InitialConditions=[0 -81.9543 0.907703 0.907703 0.907703 -8.76021 -128.76 111.24 1.25655]  SetSaturation=off  Saturation=[0.6404,0.7127,0.8441,0.9214,0.9956,1.082,1.19,1.316,1.457;0.7,0.7698,0.8872,0.9466,0.9969,1.046,1.1,1.151,1.201]  LoadFlowParameters=[1,0,0,0,0]  TsPowergui=0  TsBlock=-1  IterativeModel=Trapezoidal non iterative  IterativeDiscreteModel=Trapezoidal non iterative  BusType=PV  Pref=400e6  Qref=0  Qmin=-inf  Qmax=inf  PLF=0  QLF=0
  MPP3-TEST2 111 km : spsDistributedParametersLineLib/Distributed Parameters Line  Phases=3  Length=111  Frequency=60  Resistance=[0.01273 0.3864]/6  Inductance="[0.9337e-3  4.1264e-3]/6"  Capacitance=[12.74e-9 7.751e-9]*6  x1=[-0.00066 -2.09099101706191e-09 0 0;-0.0006 -1.58154736736312e-09 0 0;-0.00054 -1.07129456880757e-09 0 0;-0.00048 -5.60493676155357e-10 0 0;-0.00042 -4.94060245816956e-11 -26730.0800402199 -218491.44634908;-0.00036 4.61706904027061e-10 -21781.5076719494 -219040.147206954;-0.0003 9.72583614852354e-10 -16821.7914818779 -219476.78307812;-0.00024 1.48296273392901e-09 -11853.4689524533 -219801.130571598;-0.00018 1.99258314186899e-09 -6879.08196928572 -220013.023745218;-0.00012 2.50118410745488e-09 -1901.17552067184 -220112.354190517;-6e-05 3.00850542103483e-09 3077.7036044681 -220099.071088203]  x2=[-0.00066 3.23618164671738e-09 0 0;-0.0006 3.75721745049934e-09 0 0;-0.00054 4.27633099240824e-09 0 0;-0.00048 4.79325668436391e-09 0 0;-0.00042 5.30773005763066e-09 -31816.6053327474 -220884.499667418;-0.00036 5.81948789812434e-09 -26812.6065500283 -221547.633435284;-0.0003 6.32826838107758e-09 -21794.8899423582 -222097.419340155;-0.00024 6.8338112049941e-09 -16766.0226662703 -222533.576101403;-0.00018 7.33585772482384e-09 -11728.5775831858 -222855.880573169;-0.00012 7.83415108429049e-09 -6685.13194309062 -223064.167858532;-6e-05 8.32843634730394e-09 -1638.26606596631 -223158.331393866]  x3=[-0.00066 -1.93033111027684e-11 0 0;-0.0006 -1.12531525242088e-11 0 0;-0.00054 -3.19723662488356e-12 0 0;-0.00048 4.86031503977716e-12 0 0;-0.00042 1.29153800774552e-11 -1334.68845734272 -4013.2609162694;-0.00036 2.09638373680369e-11 -1243.57693857679 -4042.42216151439;-0.0003 2.90015691720539e-11 -1151.82918287042 -4069.51522888616;-0.00024 3.7024463237395e-11 -1059.49213007074 -4094.52625707085;-0.00018 4.50284149032105e-11 -966.613021520158 -4117.44244996427;-0.00012 5.30093291999321e-11 -873.239375886808 -4138.2520832187;-6e-05 6.09631229443352e-11 -779.418964853146 -4156.94451024125]  x4=[-0.00066 -1.92538466805171e-11 0 0;-0.0006 -1.89950385163193e-11 0 0;-0.00054 -1.87265121394286e-11 0 0;-0.00048 -1.84484049329013e-11 0 0;-0.00042 -1.81608591815229e-11 -659.920524240179 -5593.0489227371;-0.00036 -1.78640219990131e-11 -533.250819180359 -5606.54453752769;-0.0003 -1.75580452527595e-11 -406.308293148105 -5617.17174053585;-0.00024 -1.72430854861192e-11 -279.157892285362 -5624.92509468816;-0.00018 -1.69193038383287e-11 -151.86466908668 -5629.80063322536;-0.00012 -1.65868659620616e-11 -24.4937491171581 -5631.79586173184;-6e-05 -1.62459419386783e-11 102.889702307005 -5630.90975941184]  x5=0.000627751139365274  V1=[1.134e-27 1.175e-15 1.175e-15;377 377 377;0.8883 -1.731 2.981]  V2=[1.245e-23 7.93e-13 7.93e-13;377 377 377;-1.459 -1.742 2.971]  I1=[6.861e-26 2.027e-14 2.027e-14;377 377 377;-2.79 3.007 1.436]  I2=[6.467e-26 2.017e-14 2.017e-14;377 377 377;0.1116 -0.2797 -1.851]  nHarmo=1  Measurements=None  Decoupling=off  VsMag0=0  VrMag0=0  VsAngle0=0  VrAngle0=0  IsMag0=0  IrMag0=0  IsAngle0=0  IrAngle0=0
      settings: LibrarySourceBlock=sps_lib/Power Grid Elements/Distributed Parameters Line
  MPP3_800MVA 17KV : spsSynchronousMachinepuStandardLib/Synchronous Machine pu Standard  PresetModel=No  MechanicalLoad=Mechanical power Pm  ShowDetailedParameters=on  RotorType=Salient-pole  Units=per unit standard parameters  MeasurementBus=off  NominalParameters=[800e6 17000 60]  Reactances1=[ 1.81, 0.3, 0.23, 1.76, 0.65, 0.25, 0.15 ]  Reactances2=[ 1.305, 0.296, 0.252, 0.474, 0.243, 0.18 ]  dAxisTimeConstants=Short-circuit  qAxisTimeConstants=Open-circuit  TimeConstants1="[ 4.4849  0.0681  0.1  ]"  TimeConstants2=[ 8.0, 0.03, 1.0, 0.07 ]  TimeConstants3="[  4.49  0.0681  0.0513  ]"  TimeConstants4=[ 8.0, 0.03, 0.3371, 0.0295 ]  TimeConstants5=[ 1.01, 0.053, 0.1 ]  TimeConstants6=[ 1.3201, 0.023, 1.0, 0.07 ]  TimeConstants7=[0.012 0.003 0.003]  TimeConstants8=[ 1.3201, 0.0231, 0.3371, 0.0295 ]  StatorResistance=2.8544e-3  Mechanical=[3.5 0 32]  PolePairs=20  InitialConditions=[0 -81.9543 0.907703 0.907703 0.907703 -8.76021 -128.76 111.24 1.25655]  SetSaturation=off  Saturation=[0.6404,0.7127,0.8441,0.9214,0.9956,1.082,1.19,1.316,1.457;0.7,0.7698,0.8872,0.9466,0.9969,1.046,1.1,1.151,1.201]  LoadFlowParameters=[1,0,0,0,0]  TsPowergui=0  TsBlock=-1  IterativeModel=Trapezoidal non iterative  IterativeDiscreteModel=Trapezoidal non iterative  BusType=PV  Pref=699.2e6  Qref=0  Qmin=-inf  Qmax=inf  PLF=0  QLF=0
  MPP4-TEST2 96 km : spsDistributedParametersLineLib/Distributed Parameters Line  Phases=3  Length=96  Frequency=60  Resistance=[0.01273 0.3864]/6  Inductance="[0.9337e-3  4.1264e-3]/6"  Capacitance=[12.74e-9 7.751e-9]*6  x1=[-0.0006 6.57643468960351e-10 -23285.1371531403 -202261.418665078;-0.00054 1.716984948932e-09 -18704.5284899633 -202736.35336149;-0.00048 2.77544798767754e-09 -14114.350244391 -203107.564393386;-0.00042 3.8324910559482e-09 -9516.95083643033 -203374.861842342;-0.00036 4.88757335097835e-09 -4914.68238056876 -203538.108954044;-0.0003 5.94015507317016e-09 -309.899482388396 -203597.222208253;-0.00024 6.9896977022651e-09 4295.04196609344 -203552.171361536;-0.00018 8.03566427286079e-09 8897.78599174217 -203402.97946274;-0.00012 9.07751964913248e-09 13495.9777456653 -203149.722841195;-6e-05 1.01147307986184e-08 18087.2647079968 -202792.531067669]  x2=[-0.0006 3.75721745049934e-09 -46720.7362948807 -218218.692783999;-0.00054 4.27633099240824e-09 -41773.2171984774 -219219.60344594;-0.00048 4.79325668436391e-09 -36804.326152275 -220108.357308046;-0.00042 5.30773005763066e-09 -31816.6053327474 -220884.499667418;-0.00036 5.81948789812434e-09 -26812.6065500283 -221547.633435284;-0.0003 6.32826838107758e-09 -21794.8899423582 -222097.419340155;-0.00024 6.8338112049941e-09 -16766.0226662703 -222533.576101403;-0.00018 7.33585772482384e-09 -11728.5775831858 -222855.880573169;-0.00012 7.83415108429049e-09 -6685.13194309062 -223064.167858532;-6e-05 8.32843634730394e-09 -1638.26606596631 -223158.331393866]  x3=[-0.0006 8.81117564722618e-10 -3774.32458796234 -380.237138522721;-0.00054 8.86934341154347e-10 -3764.75865713092 -465.506118798111;-0.00048 8.9229734558848e-10 -3753.26660620578 -550.536937541561;-0.00042 8.9720383421285e-10 -3739.8543147325 -635.286091415011;-0.00036 9.01651296777216e-10 -3724.52864468725 -719.710221185356;-0.0003 9.05637457877551e-10 -3707.29743696599 -803.766133907827;-0.00024 9.09160278120179e-10 -3688.16950737301 -887.4108250243;-0.00018 9.1221795516517e-10 -3667.15464211052 -970.601500365224;-0.00012 9.1480892464845e-10 -3644.26359277189 -1053.29559804391;-6e-05 9.16931860982153e-10 -3619.50807084096 -1135.45081023197]  x4=[-0.0006 -9.06455468186357e-10 1646.95914868655 -8810.6664445221;-0.00054 -8.9984997343226e-10 1845.81297746985 -8771.16317288888;-0.00048 -8.92784098804441e-10 2043.72245422717 -8727.17241210396;-0.00042 -8.85261459334919e-10 2240.58632481325 -8678.71666865339;-0.00036 -8.77285903745051e-10 2436.30387003429 -8625.82073339089;-0.0003 -8.68861512476446e-10 2630.7749571777 -8568.51166885435;-0.00024 -8.59992595603345e-10 2823.90009124188 -8506.81879542014;-0.00018 -8.50683690627496e-10 3015.58046583971 -8440.77367630224;-0.00012 -8.40939560156695e-10 3205.7180137497 -8370.41010140399;-6e-05 -8.30765189468142e-10 3394.21545708899 -8295.76407003046]  x5=0.000542919904315913  V1=[8.106e-27 2.861e-16 2.861e-16;377 377 377;-1.836 -1.712 3.001]  V2=[1.245e-23 7.93e-13 7.93e-13;377 377 377;-1.427 -1.722 2.99]  I1=[7.942e-26 2.345e-14 2.345e-14;377 377 377;-2.756 3.026 1.455]  I2=[7.544e-26 2.335e-14 2.335e-14;377 377 377;0.1775 -0.2404 -1.811]  nHarmo=1  Measurements=None  Decoupling=off  VsMag0=0  VrMag0=0  VsAngle0=0  VrAngle0=0  IsMag0=0  IrMag0=0  IsAngle0=0  IrAngle0=0
      settings: LibrarySourceBlock=sps_lib/Power Grid Elements/Distributed Parameters Line
  MPP4_3800MVA 17KV : spsSynchronousMachinepuStandardLib/Synchronous Machine pu Standard  PresetModel=No  MechanicalLoad=Mechanical power Pm  ShowDetailedParameters=on  RotorType=Salient-pole  Units=per unit standard parameters  MeasurementBus=off  NominalParameters=[3800e6 17000 60]  Reactances1=[ 1.81, 0.3, 0.23, 1.76, 0.65, 0.25, 0.15 ]  Reactances2=[ 1.305, 0.296, 0.252, 0.474, 0.243, 0.18 ]  dAxisTimeConstants=Short-circuit  qAxisTimeConstants=Open-circuit  TimeConstants1="[ 4.4849  0.0681  0.1  ]"  TimeConstants2=[ 8.0, 0.03, 1.0, 0.07 ]  TimeConstants3="[  4.49  0.0681  0.0513  ]"  TimeConstants4=[ 8.0, 0.03, 0.3371, 0.0295 ]  TimeConstants5=[ 1.01, 0.053, 0.1 ]  TimeConstants6=[ 1.3201, 0.023, 1.0, 0.07 ]  TimeConstants7=[0.012 0.003 0.003]  TimeConstants8=[ 1.3201, 0.0231, 0.3371, 0.0295 ]  StatorResistance=2.8544e-3  Mechanical=[3.5 0 32]  PolePairs=20  InitialConditions=[0 -81.9543 0.907703 0.907703 0.907703 -8.76021 -128.76 111.24 1.25655]  SetSaturation=off  Saturation=[0.6404,0.7127,0.8441,0.9214,0.9956,1.082,1.19,1.316,1.457;0.7,0.7698,0.8872,0.9466,0.9969,1.046,1.1,1.151,1.201]  LoadFlowParameters=[1,0,0,0,0]  TsPowergui=0  TsBlock=-1  IterativeModel=Trapezoidal non iterative  IterativeDiscreteModel=Trapezoidal non iterative  BusType=PV  Pref=3200e6  Qref=0  Qmin=-inf  Qmax=inf  PLF=0  QLF=0
  MPP5_4200MVA 17KV : spsSynchronousMachinepuStandardLib/Synchronous Machine pu Standard  PresetModel=No  MechanicalLoad=Mechanical power Pm  ShowDetailedParameters=on  RotorType=Salient-pole  Units=per unit standard parameters  MeasurementBus=off  NominalParameters=[4200e6 17000 60]  Reactances1=[ 1.81, 0.3, 0.23, 1.76, 0.65, 0.25, 0.15 ]  Reactances2=[ 1.305, 0.296, 0.252, 0.474, 0.243, 0.18 ]  dAxisTimeConstants=Short-circuit  qAxisTimeConstants=Open-circuit  TimeConstants1="[ 4.4849  0.0681  0.1  ]"  TimeConstants2=[ 8.0, 0.03, 1.0, 0.07 ]  TimeConstants3="[  4.49  0.0681  0.0513  ]"  TimeConstants4=[ 8.0, 0.03, 0.3371, 0.0295 ]  TimeConstants5=[ 1.01, 0.053, 0.1 ]  TimeConstants6=[ 1.3201, 0.023, 1.0, 0.07 ]  TimeConstants7=[0.012 0.003 0.003]  TimeConstants8=[ 1.3201, 0.0231, 0.3371, 0.0295 ]  StatorResistance=2.8544e-3  Mechanical=[3.5 0 32]  PolePairs=20  InitialConditions=[0 -81.9543 0.907703 0.907703 0.907703 -8.76021 -128.76 111.24 1.25655]  SetSaturation=off  Saturation=[0.6404,0.7127,0.8441,0.9214,0.9956,1.082,1.19,1.316,1.457;0.7,0.7698,0.8872,0.9466,0.9969,1.046,1.1,1.151,1.201]  LoadFlowParameters=[1,0,0,0,0]  TsPowergui=0  TsBlock=-1  IterativeModel=Trapezoidal non iterative  IterativeDiscreteModel=Trapezoidal non iterative  BusType=PV  Pref=3700e6  Qref=0  Qmin=-inf  Qmax=inf  PLF=0  QLF=0
  MPP6-CSG 186 km : spsDistributedParametersLineLib/Distributed Parameters Line  Phases=3  Length=186  Frequency=60  Resistance=[0.01273 0.3864]/6  Inductance="[0.9337e-3  4.1264e-3]/6"  Capacitance=[12.74e-9 7.751e-9]*6  x1=[-0.00108 3.92578263450044e-08 0 0;-0.00102 3.98962910115628e-08 0 0;-0.00096 4.05143439984409e-08 0 0;-0.0009 4.11116690983104e-08 0 0;-0.00084 4.1687960708613e-08 0 0;-0.00078 4.2242923987912e-08 0 0;-0.00072 4.27762750067394e-08 0 0;-0.00066 4.32877408928586e-08 -147489.051282816 -243514.240096791;-0.0006 4.37770599708715e-08 -141943.625883865 -246787.816804634;-0.00054 4.42439818960963e-08 -136325.579503095 -249935.132305285;-0.00048 4.46882677826483e-08 -130637.786436844 -252954.576373978;-0.00042 4.51096903256584e-08 -124883.156665143 -255844.604207336;-0.00036 4.55080339175667e-08 -119064.634362917 -258603.737213716;-0.0003 4.58830947584309e-08 -113185.196393689 -261230.56376969;-0.00024 4.62346809601947e-08 -107247.850786564 -263723.739942254;-0.00018 4.65626126448605e-08 -101255.635197265 -266081.990176409;-0.00012 4.6866722036519e-08 -95211.615354009 -268304.10794776;-6e-05 4.71468535471862e-08 -89118.88348903 -270388.956379794]  x2=[-0.00108 3.05196608822481e-08 0 0;-0.00102 3.16410903132648e-08 0 0;-0.00096 3.27463315778171e-08 0 0;-0.0009 3.38348192140516e-08 0 0;-0.00084 3.49059963315806e-08 0 0;-0.00078 3.59593148963977e-08 0 0;-0.00072 3.69942360112621e-08 0 0;-0.00066 3.80102301914082e-08 -159481.256217259 -255955.058250877;-0.0006 3.90067776354401e-08 -153651.381927409 -259496.688343458;-0.00054 3.99833684912713e-08 -147742.896751414 -262905.555135335;-0.00048 4.09395031169747e-08 -141758.823579467 -266179.914587269;-0.00042 4.18746923364084e-08 -135702.223973974 -269318.091476461;-0.00036 4.27884576894874e-08 -129576.196603207 -272318.480253627;-0.0003 4.36803316769727e-08 -123383.875655965 -275179.545864429;-0.00024 4.45498579996524e-08 -117128.429238066 -277899.824534833;-0.00018 4.53965917917926e-08 -110813.057751484 -280477.924520007;-0.00012 4.62200998487397e-08 -104440.992256967 -282912.52681636;-6e-05 4.70199608485549e-08 -98015.492820963 -285202.385836371]  x3=[-0.00108 -1.8924987456685e-10 0 0;-0.00102 -1.84393953029028e-10 0 0;-0.00096 -1.79443692137628e-10 0 0;-0.0009 -1.74401624537593e-10 0 0;-0.00084 -1.69270329843872e-10 0 0;-0.00078 -1.64052433321647e-10 0 0;-0.00072 -1.58750604543194e-10 0 0;-0.00066 -1.53367556022083e-10 -5084.54143659808 -3903.49127599412;-0.0006 -1.47906041825405e-10 -4994.95307859977 -4017.49316245418;-0.00054 -1.42368856164739e-10 -4902.80921031034 -4129.43962517759;-0.00048 -1.36758831966585e-10 -4808.15697423542 -4239.27339028549;-0.00042 -1.31078839422985e-10 -4711.04479620795 -4346.93826479415;-0.00036 -1.25331784523077e-10 -4611.52236061264 -4452.37916536436;-0.0003 -1.19520607566343e-10 -4509.64058496651 -4555.54214648306;-0.00024 -1.1364828165829e-10 -4405.45159386853 -4656.37442806288;-0.00018 -1.07717811189362e-10 -4299.00869233174 -4754.8244224454;-0.00012 -1.01732230297834e-10 -4190.3663385114 -4850.84176079434;-6e-05 -9.56946013174893e-11 -4079.58011584322 -4944.3773188652]  x4=[-0.00108 6.0278554322305e-10 0 0;-0.00102 6.13890005488892e-10 0 0;-0.00096 6.24680390284542e-10 0 0;-0.0009 6.35151177049757e-10 0 0;-0.00084 6.45297008736548e-10 0 0;-0.00078 6.55112694549952e-10 0 0;-0.00072 6.64593212603734e-10 0 0;-0.00066 6.73733712489677e-10 -3013.48635092652 -6270.5217032714;-0.0006 6.82529517759142e-10 -2870.89168841968 -6337.07602944636;-0.00054 6.90976128315627e-10 -2726.82822467706 -6400.38819042895;-0.00048 6.99069222717095e-10 -2581.3696652287 -6460.42579454774;-0.00042 7.06804660386906e-10 -2434.59042936138 -6517.1581254551;-0.00036 7.14178483732215e-10 -2286.56561204434 -6570.55615784224;-0.0003 7.21186920168745e-10 -2137.37094550931 -6620.59257228911;-0.00024 7.27826384050915e-10 -1987.08276050448 -6667.24176924151;-0.00018 7.34093478506319e-10 -1835.7779472423 -6710.4798821083;-0.00012 7.39984997173632e-10 -1683.53391606105 -6750.284789472;-6e-05 7.4549792584304e-10 -1530.4285578202 -6786.63612640648]  x5=0.00105190731461208  V1=[8.574e-27 4.511e-17 4.511e-17;377 377 377;-2.265 1.301 -0.2697]  V2=[1.073e-22 6.76e-12 6.76e-12;377 377 377;0.1921 1.269 -0.3021]  I1=[3.519e-25 1.037e-13 1.037e-13;377 377 377;-1.143 -0.2664 -1.837]  I2=[3.187e-25 1.028e-13 1.028e-13;377 377 377;1.591 2.633 1.062]  nHarmo=1  Measurements=None  Decoupling=off  VsMag0=0  VrMag0=0  VsAngle0=0  VrAngle0=0  IsMag0=0  IrMag0=0  IsAngle0=0  IrAngle0=0
      settings: LibrarySourceBlock=sps_lib/Power Grid Elements/Distributed Parameters Line
  MPP6_490MVA 17KV : spsSynchronousMachinepuStandardLib/Synchronous Machine pu Standard  PresetModel=No  MechanicalLoad=Mechanical power Pm  ShowDetailedParameters=on  RotorType=Salient-pole  Units=per unit standard parameters  MeasurementBus=off  NominalParameters=[490e6 13800 60]  Reactances1=[ 1.81, 0.3, 0.23, 1.76, 0.65, 0.25, 0.15 ]  Reactances2=[ 1.305, 0.296, 0.252, 0.474, 0.243, 0.18 ]  dAxisTimeConstants=Short-circuit  qAxisTimeConstants=Open-circuit  TimeConstants1="[ 4.4849  0.0681  0.1  ]"  TimeConstants2=[ 8.0, 0.03, 1.0, 0.07 ]  TimeConstants3="[  4.49  0.0681  0.0513  ]"  TimeConstants4=[ 8.0, 0.03, 0.3371, 0.0295 ]  TimeConstants5=[ 1.01, 0.053, 0.1 ]  TimeConstants6=[ 1.3201, 0.023, 1.0, 0.07 ]  TimeConstants7=[0.012 0.003 0.003]  TimeConstants8=[ 1.3201, 0.0231, 0.3371, 0.0295 ]  StatorResistance=2.8544e-3  Mechanical=[3.5 0 32]  PolePairs=20  InitialConditions=[0 -81.9543 0.907703 0.907703 0.907703 -8.76021 -128.76 111.24 1.25655]  SetSaturation=off  Saturation=[0.6404,0.7127,0.8441,0.9214,0.9956,1.082,1.19,1.316,1.457;0.7,0.7698,0.8872,0.9466,0.9969,1.046,1.1,1.151,1.201]  LoadFlowParameters=[1,0,0,0,0]  TsPowergui=0  TsBlock=-1  IterativeModel=Trapezoidal non iterative  IterativeDiscreteModel=Trapezoidal non iterative  BusType=PV  Pref=415e6  Qref=0  Qmin=-inf  Qmax=inf  PLF=0  QLF=0
  PNS-CON 260 km : spsDistributedParametersLineLib/Distributed Parameters Line  Phases=3  Length=271  Frequency=60  Resistance=[0.01273 0.3864]/6  Inductance="[0.9337e-3  4.1264e-3]/6"  Capacitance=[12.74e-9 7.751e-9]*6  x1=[-0.00156 1.46713520016474e-08 -222746.66543221 -201982.240584507;-0.0015 1.58628123780612e-08 -218121.329379785 -206968.582830171;-0.00144 1.70461570465513e-08 -213384.398424831 -211849.03612452;-0.00138 1.82207805861197e-08 -208538.296068753 -216621.103537466;-0.00132 1.93860820376588e-08 -203585.501667061 -221282.343591146;-0.00126 2.05414652114139e-08 -198528.549160888 -225830.371509016;-0.0012 2.16863389920042e-08 -193370.025780579 -230262.860435957;-0.00114 2.28201176408487e-08 -188112.570722014 -234577.542628731;-0.00108 2.39422210958409e-08 -182758.873796346 -238772.210616201;-0.00102 2.5052075268119e-08 -177311.674053849 -242844.718328717;-0.00096 2.61491123357809e-08 -171773.758382562 -246792.982196081;-0.0009 2.72327710343917e-08 -166147.960082473 -250614.982213544;-0.00084 2.83024969441376e-08 -160437.157415945 -254308.762975274;-0.00078 2.93577427734768e-08 -154644.272135144 -257872.43467478;-0.00072 3.03979686391444e-08 -148772.267987222 -261304.174071771;-0.00066 3.14226423423664e-08 -142824.149198002 -264602.225424962;-0.0006 3.24312396411423e-08 -136802.958934965 -267764.901390338;-0.00054 3.34232445184574e-08 -130711.777750309 -270790.583884437;-0.00048 3.43981494462864e-08 -124553.722004881 -273677.724912185;-0.00042 3.53554556452538e-08 -118331.942273786 -276424.847358886;-0.00036 3.62946733398195e-08 -112049.621734501 -279030.545745933;-0.0003 3.7215322008856e-08 -105709.974538298 -281493.486949886;-0.00024 3.81169306314928e-08 -99316.2441658255 -283812.410884513;-0.00018 3.89990379280986e-08 -92871.7017676844 -285986.131145481;-0.00012 3.98611925962809e-08 -86379.6444908473 -288013.53561734;-6e-05 4.07029535417809e-08 -79843.3937917763 -289893.587042498]  x2=[-0.00156 8.09868005871819e-09 -257078.982867692 -218326.683846464;-0.0015 8.8698925663467e-09 -252075.190293638 -224085.36071323;-0.00144 9.6365670730415e-09 -246942.431394416 -229729.391368834;-0.00138 1.03983113339584e-08 -241683.33218432 -235255.888222902;-0.00132 1.11547356266582e-08 -236300.583315685 -240662.023817527;-0.00126 1.19054529504956e-08 -230796.938702293 -245945.032273843;-0.0012 1.2650079224616e-08 -225175.214110424 -251102.210707107;-0.00114 1.33882334844586e-08 -219438.285718256 -256130.920609538;-0.00108 1.41195380766643e-08 -213589.088644361 -261028.589200229;-0.00102 1.4843618852291e-08 -207630.615446043 -265792.710741432;-0.00096 1.55601053582343e-08 -201565.914588291 -270420.847820535;-0.0009 1.62686310267587e-08 -195398.088884125 -274910.63259709;-0.00084 1.696883336304e-08 -189130.293907145 -279259.768014244;-0.00078 1.76603541306248e-08 -182765.736377075 -283466.028973955;-0.00072 1.83428395347105e-08 -176307.672519153 -287527.263475393;-0.00066 1.90159404031536e-08 -169759.406398179 -291441.393715943;-0.0006 1.96793123651122e-08 -163124.288228098 -295206.417154251;-0.00054 2.0332616027233e-08 -156405.712657969 -298820.407534756;-0.00048 2.09755171472907e-08 -149607.117035199 -302281.515873199;-0.00042 2.16076868051928e-08 -142731.979646933 -305587.971402601;-0.00036 2.22288015712613e-08 -135783.817940495 -308738.082479218;-0.0003 2.28385436717049e-08 -128766.186723802 -311730.237448014;-0.00024 2.34366011511983e-08 -121682.676346656 -314562.905467219;-0.00018 2.40226680324841e-08 -114536.910863854 -317234.637291533;-0.00012 2.45964444729166e-08 -107332.546181055 -319744.066013586;-6e-05 2.51576369178668e-08 -100073.268184352 -322089.907763276]  x3=[-0.00156 2.14672674772384e-10 -6799.95613303636 -1408.91800798249;-0.0015 2.20881434329114e-10 -6766.34974352875 -1562.35628354046;-0.00144 2.26977186862622e-10 -6729.28156446457 -1714.99522875475;-0.00138 2.32956813673275e-10 -6688.77056060918 -1866.75675072054;-0.00132 2.38817255473505e-10 -6644.83745814072 -2017.56320543896;-0.00126 2.44555513953e-10 -6597.5047340462 -2167.3374375412;-0.0012 2.5016865331269e-10 -6546.79660462186 -2316.0028197626;-0.00114 2.55653801766761e-10 -6492.73901308371 -2463.4832921466;-0.00108 2.61008153011908e-10 -6435.35961629445 -2609.7034009584;-0.00102 2.66228967663098e-10 -6374.68777061371 -2754.58833728849;-0.00096 2.71313574655086e-10 -6310.75451687884 -2898.06397532628;-0.0009 2.76259372608982e-10 -6243.5925645238 -3040.05691028424;-0.00084 2.81063831163165e-10 -6173.23627484442 -3180.4944959531;-0.00078 2.85724492267862e-10 -6099.72164341854 -3319.30488186905;-0.00072 2.90238971442734e-10 -6023.08628169 -3456.41705007373;-0.00066 2.94604958996816e-10 -5943.3693977259 -3591.76085144835;-0.0006 2.98820221210201e-10 -5860.61177615708 -3725.26704160326;-0.00054 3.02882601476852e-10 -5774.85575731193 -3856.86731630467;-0.00048 3.06790021407961e-10 -5686.14521555427 -3986.49434642033;-0.00042 3.1054048189529e-10 -5594.52553683645 -4114.08181236643;-0.00036 3.14132064133953e-10 -5500.04359547904 -4239.56443803783;-0.0003 3.17562930604111e-10 -5402.74773018906 -4362.87802420458;-0.00024 3.20831326011085e-10 -5302.68771932902 -4483.95948135743;-0.00018 3.23935578183389e-10 -5199.91475544937 -4602.74686198558;-0.00012 3.26874098928254e-10 -5094.48141909745 -4719.17939227015;-6e-05 3.29645384844169e-10 -4986.44165191632 -4833.19750317723]  x4=[-0.00156 -2.44677998067204e-10 -5380.20300248226 -5935.76925307278;-0.0015 -2.3524644466273e-10 -5244.57390867991 -6055.93861434433;-0.00144 -2.25694534830312e-10 -5106.2615939573 -6173.0096455199;-0.00138 -2.16027155503519e-10 -4965.33682145035 -6286.92245089673;-0.00132 -2.06249252692247e-10 -4821.87169087668 -6397.6187505787;-0.00126 -1.96365828952251e-10 -4675.939601648 -6505.04191029348;-0.0012 -1.86381940825739e-10 -4527.6152153177 -6609.13697036759;-0.00114 -1.76302696254358e-10 -4376.97441738252 -6709.85067384486;-0.00108 -1.66133251965874e-10 -4224.09427845823 -6807.1314937336;-0.00102 -1.55878810835895e-10 -4069.05301484879 -6900.92965936882;-0.00096 -1.45544619225983e-10 -3911.92994852949 -6991.19718187579;-0.0009 -1.3513596429952e-10 -3752.80546656438 -7077.88787872204;-0.00084 -1.24658171316695e-10 -3591.7609799787 -7160.9573973452;-0.00078 -1.14116600910007e-10 -3428.87888210754 -7240.3632378446;-0.00072 -1.03516646341661e-10 -3264.24250644191 -7316.06477472499;-0.00066 -9.28637307442788e-11 -3097.93608399371 -7388.0232776813;-0.0006 -8.21633043463233e-11 -2930.04470020167 -7456.20193141378;-0.00054 -7.14208416836609e-11 -2760.6542514 -7520.56585446337;-0.00048 -6.06418387986878e-11 -2589.85140087229 -7581.08211705773;-0.00042 -4.98318104284529e-11 -2417.72353451294 -7637.71975795872;-0.00036 -3.89962871832169e-11 -2244.35871611894 -7690.44980030271;-0.0003 -2.81408127168893e-11 -2069.84564233479 -7739.24526642568;-0.00024 -1.72709408907934e-11 -1894.27359727368 -7784.08119166554;-0.00018 -6.39223293220747e-12 -1717.73240683805 -7824.93463713447;-0.00012 4.48974541086149e-12 -1540.31239276303 -7861.78470145486;-6e-05 1.53694267172173e-11 -1362.10432640618 -7894.61253145292]  x5=0.00153261764655846  V1=[1.516e-17 3.586e-06 3.586e-06;377 377 377;3.054 -1.986 2.727]  V2=[2.167e-13 0.2213 0.2213;377 377 377;-0.8435 -2.017 2.695]  I1=[4.914e-16 0.002352 0.002352;377 377 377;-2.188 2.73 1.159]  I2=[4.262e-16 0.002322 0.002322;377 377 377;0.3532 -0.7649 -2.336]  nHarmo=1  Measurements=None  Decoupling=off  VsMag0=0  VrMag0=0  VsAngle0=0  VrAngle0=0  IsMag0=0  IrMag0=0  IsAngle0=0  IrAngle0=0
      settings: LibrarySourceBlock=sps_lib/Power Grid Elements/Distributed Parameters Line
  PNS3 : spsThreePhaseVIMeasurementLib/Three-Phase V-I Measurement  VoltageMeasurement=no  SetLabelV=off  LabelV=Vabc  Vpu=off  VpuLL=off  CurrentMeasurement=no  SetLabelI=off  LabelI=Iabc  Ipu=off  Pbase=100e6  Vbase=500e3  OutputType=Complex  PhasorSimulation=off  PSBequivalent=0
  Regulators 1 : Subsystem
  Regulators 2 : Subsystem
  Regulators 3 : Subsystem
  Regulators 4 : Subsystem
  Regulators 5 : Subsystem
  Regulators 6 : Subsystem
  TEST 1 : spsThreePhaseVIMeasurementLib/Three-Phase V-I Measurement  VoltageMeasurement=no  SetLabelV=off  LabelV=Vabc  Vpu=off  VpuLL=off  CurrentMeasurement=no  SetLabelI=off  LabelI=Iabc  Ipu=off  Pbase=100e6  Vbase=500e3  OutputType=Complex  PhasorSimulation=off  PSBequivalent=0
  TEST1-MPP2 187 km : spsDistributedParametersLineLib/Distributed Parameters Line  Phases=3  Length=187  Frequency=60  Resistance=[0.01273 0.3864]/6  Inductance="[0.9337e-3  4.1264e-3]/6"  Capacitance=[12.74e-9 7.751e-9]*6  x1=[-0.00108 1.81240511066336e-08 0 0;-0.00102 1.87463792242092e-08 0 0;-0.00096 1.93591163477804e-08 0 0;-0.0009 1.99619489897128e-08 0 0;-0.00084 2.05545687296876e-08 0 0;-0.00078 2.11366723724956e-08 0 0;-0.00072 2.17079621031569e-08 0 0;-0.00066 2.22681456392893e-08 147235.445162185 224809.224771138;-0.0006 2.28169363806446e-08 152282.439097325 221421.62580843;-0.00054 2.33540535557391e-08 157251.522522768 217920.743450558;-0.00048 2.38792223655011e-08 162140.153163614 214308.368813623;-0.00042 2.43921741238637e-08 166945.829906095 210586.35005524;-0.00036 2.48926463952289e-08 171666.094077193 206756.591428981;-0.0003 2.53803831287352e-08 176298.530702536 202821.052310123;-0.00024 2.58551347892572e-08 180840.769741949 198781.746193202;-0.00018 2.6316658485073e-08 185290.487302009 194640.739661864;-0.00012 2.6764718092132e-08 189645.40682499 190400.151331568;-6e-05 2.71990843748599e-08 193903.300253596 186062.15076566]  x2=[-0.00108 2.85521483249331e-08 0 0;-0.00102 2.97448561056187e-08 0 0;-0.00096 3.09223458682989e-08 0 0;-0.0009 3.20840151874537e-08 0 0;-0.00084 3.32292697315941e-08 0 0;-0.00078 3.43575235673335e-08 0 0;-0.00072 3.54681994591619e-08 0 0;-0.00066 3.65607291647699e-08 148642.580747898 233311.037408028;-0.0006 3.76345537257727e-08 153881.505637069 229889.437791437;-0.00054 3.86891237536827e-08 159041.701904552 226350.222490604;-0.00048 3.97238997109876e-08 164120.529498588 222695.202233474;-0.00042 4.0738352187187e-08 169115.389997133 218926.246995947;-0.00036 4.17319621696493e-08 174023.727937263 215045.285045165;-0.0003 4.27042213091476e-08 178843.032122592 211054.301952973;-0.00024 4.36546321799409e-08 183570.836908047 206955.339580068;-0.00018 4.4582708534266e-08 188204.723461341 202750.495031338;-0.00012 4.54879755511113e-08 192742.321000489 198441.919582952;-6e-05 4.63699700791435e-08 197181.308006745 194031.817581722]  x3=[-0.00108 -3.39279307601412e-10 0 0;-0.00102 -3.26688119867639e-10 0 0;-0.00096 -3.13929792455239e-10 0 0;-0.0009 -3.01010852760263e-10 0 0;-0.00084 -2.87937910350975e-10 0 0;-0.00078 -2.74717653586269e-10 0 0;-0.00072 -2.61356846193791e-10 0 0;-0.00066 -2.4786232380948e-10 1861.97603725863 5503.11393838881;-0.0006 -2.3424099048034e-10 1985.96725731182 5459.59300602824;-0.00054 -2.20499815132193e-10 2108.94241981971 5413.27884500411;-0.00048 -2.06645828004258e-10 2230.83860841685 5364.19515049699;-0.00042 -1.92686117052339e-10 2351.59345876076 5312.36703463194;-0.00036 -1.78627824322506e-10 2471.14519043872 5257.82101363071;-0.0003 -1.64478142297087e-10 2589.43263857573 5200.58499424555;-0.00024 -1.50244310214862e-10 2706.39528512764 5140.68825948158;-0.00018 -1.35933610367336e-10 2821.97328984324 5078.16145361505;-0.00012 -1.21553364372981e-10 2936.10752087969 5013.03656651522;-6e-05 -1.07110929431365e-10 3048.73958505543 4945.3469172777]  x4=[-0.00108 5.68584402933913e-10 0 0;-0.00102 5.71469101740088e-10 0 0;-0.00096 5.74061426394279e-10 0 0;-0.0009 5.7636005061529e-10 0 0;-0.00084 5.78363798384498e-10 0 0;-0.00078 5.80071644547518e-10 0 0;-0.00072 5.81482715338696e-10 0 0;-0.00066 5.82596288828141e-10 3417.27694212318 5380.89365586736;-0.0006 5.8341179529108e-10 3538.10596920736 5302.22706418496;-0.00054 5.83928817499338e-10 3657.124835901 5220.84775516264;-0.00048 5.84147090934799e-10 3774.2726499527 5136.7973639586;-0.00042 5.84066503924741e-10 3889.48947637615 5050.11889230606;-0.00036 5.83687097698966e-10 4002.71636811397 4960.85668651275;-0.0003 5.83009066368712e-10 4113.89539619618 4869.05641477253;-0.00024 5.82032756827334e-10 4222.96967937765 4774.76504380069;-0.00018 5.80758668572834e-10 4329.88341323963 4678.03081480492;-0.00012 5.79187453452307e-10 4434.58189874036 4578.90321880423;-6e-05 5.77319915328439e-10 4537.01157020004 4477.4329713084]  x5=0.00105756273028204  V1=[5.148e-22 3.64e-12 3.64e-12;377 377 377;-2.284 2.392 -2.32]  V2=[4.457e-19 3.159e-07 3.159e-07;377 377 377;1.876 2.36 -2.352]  I1=[1.453e-21 4.823e-09 4.823e-09;377 377 377;0.5394 0.8251 2.396]  I2=[1.317e-21 4.781e-09 4.781e-09;377 377 377;-3.011 -2.56 -0.9894]  nHarmo=1  Measurements=None  Decoupling=off  VsMag0=0  VrMag0=0  VsAngle0=0  VrAngle0=0  IsMag0=0  IrMag0=0  IsAngle0=0  IrAngle0=0
      settings: LibrarySourceBlock=sps_lib/Power Grid Elements/Distributed Parameters Line
  TEST1-PNS 235 km : spsDistributedParametersLineLib/Distributed Parameters Line  Phases=3  Length=235  Frequency=60  Resistance=[0.01273 0.3864]/6  Inductance="[0.9337e-3  4.1264e-3]/6"  Capacitance=[12.74e-9 7.751e-9]*6  x1=[-0.00138 2.23819514632633e-08 -188845.979573234 -202152.714326624;-0.00132 2.36414514535038e-08 -184225.463426501 -206372.261490083;-0.00126 2.4888856040337e-08 -179510.694128583 -210486.224791243;-0.0012 2.61235270285267e-08 -174704.083842573 -214492.499450462;-0.00114 2.73448327375814e-08 -169808.091719109 -218389.035783596;-0.00108 2.85521483249331e-08 -164825.222638229 -222173.840250658;-0.00102 2.97448561056187e-08 -159758.025927827 -225844.976475747;-0.00096 3.09223458682989e-08 -154609.094059372 -229400.566237736;-0.0009 3.20840151874537e-08 -149381.061321548 -232838.790431202;-0.00084 3.32292697315941e-08 -144076.602472507 -236157.889997117;-0.00078 3.43575235673335e-08 -138698.431371412 -239356.166822814;-0.00072 3.54681994591619e-08 -133249.299589975 -242431.984610771;-0.00066 3.65607291647699e-08 -127731.995004704 -245383.769715774;-0.0006 3.76345537257727e-08 -122149.340370573 -248210.011950018;-0.00054 3.86891237536827e-08 -116504.191876847 -250909.265355756;-0.00048 3.97238997109876e-08 -110799.437685808 -253480.148945067;-0.00042 4.0738352187187e-08 -105037.99645511 -255921.347406403;-0.00036 4.17319621696493e-08 -99222.8158445467 -258231.611777524;-0.0003 4.27042213091476e-08 -93356.8710079705 -260409.760084487;-0.00024 4.36546321799409e-08 -87443.1630711501 -262454.677946373;-0.00018 4.4582708534266e-08 -81484.7175963385 -264365.319145416;-0.00012 4.54879755511113e-08 -75484.5830343402 -266140.706162274;-6e-05 4.63699700791435e-08 -69445.8291648668 -267779.930676146]  x2=[-0.00138 1.59387661717287e-08 -236084.151867817 -235659.396095287;-0.00132 1.70606685559652e-08 -230693.709587248 -240938.788578156;-0.00126 1.81738423869236e-08 -225185.240142124 -246094.91232475;-0.0012 1.92777181443029e-08 -219561.561767199 -251125.129366889;-0.00114 2.03717310648683e-08 -213825.551640242 -256026.866152584;-0.00108 2.14553214313945e-08 -207980.144410025 -260797.614862723;-0.00102 2.25279348590277e-08 -202028.330694896 -265434.934694113;-0.00096 2.35890225789187e-08 -195973.155552729 -269936.453108239;-0.0009 2.46380417189832e-08 -189817.716923014 -274299.867045103;-0.00084 2.56744555816457e-08 -183565.164041892 -278522.944101508;-0.00078 2.66977339184232e-08 -177218.695830953 -282603.523673198;-0.00072 2.77073532012106e-08 -170781.559260602 -286539.518060265;-0.00066 2.87027968901272e-08 -164257.047688852 -290328.91353525;-0.0006 2.96835556977882e-08 -157648.499176384 -293969.771373409;-0.00054 3.06491278498651e-08 -150959.294778728 -297460.228844597;-0.00048 3.15990193418033e-08 -144192.856816455 -300798.500166274;-0.00042 3.25327441915635e-08 -137352.647124258 -303982.87741715;-0.00036 3.34498246882592e-08 -130442.165279807 -307011.731410981;-0.0003 3.43497916365628e-08 -123464.946813305 -309883.512530098;-0.00024 3.52321845967539e-08 -116424.561398643 -312596.751518215;-0.00018 3.60965521202894e-08 -109324.611027091 -315150.060232132;-0.00012 3.69424519807725e-08 -102168.728164451 -317542.13235193;-6e-05 3.77694514002043e-08 -94960.5738926214 -319771.744049313]  x3=[-0.00138 1.28546645006303e-10 -7411.15882909501 -432.40192406485;-0.00132 1.36260846218105e-10 -7399.48237499685 -599.913827454954;-0.00126 1.43905333863172e-10 -7384.02020898893 -767.118803845798;-0.0012 1.51476196880369e-10 -7364.78024180109 -933.931308081869;-0.00114 1.58969561876283e-10 -7341.77231695604 -1100.26599580366;-0.00108 1.66381595106922e-10 -7315.00820573329 -1266.03776711142;-0.00102 1.73708504439126e-10 -7284.50160114667 -1431.16181010383;-0.00096 1.80946541290695e-10 -7250.26811093879 -1595.55364426937;-0.0009 1.88092002548232e-10 -7212.32524959581 -1759.12916370806;-0.00084 1.95141232461724e-10 -7170.69242938668 -1921.80468016163;-0.00078 2.02090624514894e-10 -7125.39095043152 -2083.49696582995;-0.00072 2.08936623270356e-10 -7076.44398980403 -2244.12329595196;-0.00066 2.15675726188649e-10 -7023.8765896737 -2403.60149112913;-0.0006 2.22304485420194e-10 -6967.71564449379 -2561.84995936999;-0.00054 2.28819509569283e-10 -6907.98988724156 -2718.7877378341;-0.00048 2.35217465429179e-10 -6844.72987471805 -2874.3345342541;-0.00042 2.41495079687442e-10 -6777.96797191457 -3028.41076801479;-0.00036 2.47649140600621e-10 -6707.7383354542 -3180.93761086796;-0.0003 2.53676499637438e-10 -6634.07689611667 -3331.83702726244;-0.00024 2.59574073089638e-10 -6557.02134045543 -3481.03181426851;-0.00018 2.65338843649669e-10 -6476.61109151659 -3628.44564107632;-0.00012 2.70967861954389e-10 -6392.88728866932 -3774.00308804819;-6e-05 2.76458248094024e-10 -6305.8927665582 -3917.62968530466]  x4=[-0.00138 -4.88054613148759e-11 -3414.19519615842 -7748.08792207673;-0.00132 -3.69895677852774e-11 -3238.07911636093 -7823.32752143662;-0.00126 -2.51547497093114e-11 -3060.30637545469 -7894.56456187806;-0.0012 -1.33070619985877e-11 -2880.96792525881 -7961.76259721486;-0.00114 -1.45256614905944e-12 -2700.15551863819 -8024.88724769047;-0.00108 1.04026728601512e-11 -2517.9616625611 -8083.9062175673;-0.00102 2.22525896697071e-11 -2334.47957077087 -8138.78931164981;-0.00096 3.40911216432075e-11 -2149.803116096 -8189.50845073294;-0.0009 4.59122119689437e-11 -1964.02678242315 -8236.03768596796;-0.00084 5.77098127586765e-11 -1777.24561635737 -8278.35321213835;-0.00078 6.94778881418472e-11 -1589.55517859453 -8316.43337983904;-0.00072 8.12104173536408e-11 -1401.05149503073 -8350.25870655259;-0.00066 9.29013978153202e-11 -1211.83100763361 -8379.81188661682;-0.0006 1.04544848205257e-10 -1021.99052510092 -8405.07780007873;-0.00054 1.16134811519085e-10 -831.627173331376 -8426.04352043015;-0.00048 1.27665358117416e-10 -640.838345733254 -8442.69832122113;-0.00042 1.39130588759549e-10 -449.721653396123 -8455.03368154784;-0.00036 1.50524637621635e-10 -258.374875151215 -8463.04329041202;-0.0003 1.61841675297738e-10 -66.8959075459598 -8466.72304994976;-0.00024 1.73075911782268e-10 124.61728524169 -8466.0710775281;-0.00018 1.84221599432256e-10 316.066721523547 -8461.08770670816;-0.00012 1.9527303590795e-10 507.354452230431 -8451.77548707455;-6e-05 2.06224567090243e-10 698.382611024722 -8438.13918293089]  x5=0.00132902268243999  V1=[4.457e-19 3.159e-07 3.159e-07;377 377 377;1.774 1.251 -0.3202]  V2=[2.934e-17 4.144e-06 4.144e-06;377 377 377;-1.608 -1.933 2.78]  I1=[7.734e-20 5.426e-08 5.426e-08;377 377 377;-2.952 2.797 1.226]  I2=[6.83e-20 5.366e-08 5.366e-08;377 377 377;-0.313 -0.6082 -2.179]  nHarmo=1  Measurements=None  Decoupling=off  VsMag0=0  VrMag0=0  VsAngle0=0  VrAngle0=0  IsMag0=0  IrMag0=0  IsAngle0=0  IrAngle0=0
      settings: LibrarySourceBlock=sps_lib/Power Grid Elements/Distributed Parameters Line
  TEST2 : spsThreePhaseVIMeasurementLib/Three-Phase V-I Measurement  VoltageMeasurement=no  SetLabelV=off  LabelV=Vabc  Vpu=off  VpuLL=off  CurrentMeasurement=no  SetLabelI=off  LabelI=Iabc  Ipu=off  Pbase=100e6  Vbase=500e3  OutputType=Complex  PhasorSimulation=off  PSBequivalent=0
  CON-a : PMIOPort  Side=Left
  CON-b : PMIOPort  Port=2  Side=Left
  CON-c : PMIOPort  Port=3  Side=Left
  SAT-a : PMIOPort  Port=4  Side=Left
  SAT-b : PMIOPort  Port=5  Side=Left
  SAT-c : PMIOPort  Port=6  Side=Left
  wires:
  Regulators 1/2(Vf) -> MPP1_3700MVA 17KV/2
  Regulators 1/1(Pm) -> MPP1_3700MVA 17KV/1
  Regulators 4/1(Pm) -> MPP4_3800MVA 17KV/1
  Regulators 4/2(Vf) -> MPP4_3800MVA 17KV/2
  MPP1_3700MVA 17KV/1 -> Regulators 1/1(m)
  Regulators 3/1(Pm) -> MPP3_800MVA 17KV/1
  Regulators 2/1(Pm) -> MPP2_500MVA 17KV/1
  MPP4_3800MVA 17KV/1 -> Regulators 4/1(m)
  MPP3_800MVA 17KV/1 -> Regulators 3/1(m)
  Regulators 3/2(Vf) -> MPP3_800MVA 17KV/2
  Regulators 2/2(Vf) -> MPP2_500MVA 17KV/2
  MPP2_500MVA 17KV/1 -> Regulators 2/1(m)
  Regulators 5/1(Pm) -> MPP5_4200MVA 17KV/1
  Regulators 5/2(Vf) -> MPP5_4200MVA 17KV/2
  MPP5_4200MVA 17KV/1 -> Regulators 5/1(m)
  Regulators 6/1(Pm) -> MPP6_490MVA 17KV/1
  Regulators 6/2(Vf) -> MPP6_490MVA 17KV/2
  MPP6_490MVA 17KV/1 -> Regulators 6/1(m)
  connections:
  CLP-CSG 103 km/LConn3 -- Cs CSGN/LConn3
  CLP-TEST2 288 km/RConn1 -- Cs CLPS/LConn1 -- Cs AND/RConn1
  CLP 1/LConn3 -- 4200 MVA 17KV :650KV Transformer/RConn3 -- Cs CLPN/RConn3 -- Cs CLPS/RConn3
  "500 MVA 17KV :650KV Transformer "/LConn3 -- 1980 MVar/LConn3 -- TEST1-MPP2 187 km/LConn1
  CLP-CSG 103 km/RConn1 -- 990 MVar3/LConn1 -- CLP 1/RConn1 -- Load Flow Bus7/LConn1
  MPP3-TEST2 111 km/RConn2 -- 660 MVar4/LConn2 -- MPP4-TEST2 96 km/RConn2 -- TEST2/LConn2
  MPP2_500MVA 17KV/RConn2 -- 25 MW/LConn2 -- "500 MVA 17KV :650KV Transformer "/RConn2
  TEST1-PNS 235 km/LConn2 -- TEST 1/LConn2 -- TEST1-MPP2 187 km/RConn2
  "3700 MVA 17KV :650KV Transformer "/LConn3 -- MPP1_3700MVA 17KV/RConn3 -- 185 MW/LConn3
  "500 MVA 17KV :650KV Transformer "/RConn3 -- 25 MW/LConn3 -- MPP2_500MVA 17KV/RConn3
  40 MW/LConn1 -- MPP3_800MVA 17KV/RConn1 -- 800 MVA 17KV :650KV Transformer/RConn1 -- Load Flow Bus4/LConn1
  MPP4_3800MVA 17KV/RConn1 -- 190 MW/LConn1 -- Load Flow Bus6/LConn1 -- 3800 MVA 17KV :650KV Transformer/RConn1
  "500 MVA 17KV :650KV Transformer "/LConn1 -- 1980 MVar/LConn1 -- TEST1-MPP2 187 km/LConn3
  CLP 1/RConn3 -- 990 MVar3/LConn3 -- CLP-CSG 103 km/RConn3
  Cs CSGN/LConn2 -- CLP-CSG 103 km/LConn2
  MPP4_3800MVA 17KV/RConn3 -- 190 MW/LConn3 -- 3800 MVA 17KV :650KV Transformer/RConn3
  "3700 MVA 17KV :650KV Transformer "/LConn1 -- Load Flow Bus/LConn1 -- 185 MW/LConn1 -- MPP1_3700MVA 17KV/RConn1
  CLP 1/LConn1 -- 4200 MVA 17KV :650KV Transformer/RConn1 -- Cs CLPN/RConn1 -- Cs CLPS/RConn1
  CLP 1/LConn2 -- 4200 MVA 17KV :650KV Transformer/RConn2 -- Cs CLPN/RConn2 -- Cs CLPS/RConn2
  3800 MVA 17KV :650KV Transformer/LConn2 -- MPP4-TEST2 96 km/LConn2
  "3700 MVA 17KV :650KV Transformer "/RConn1 -- MPP1-CLP 310 km/LConn1 -- Cs MPP1D/RConn1 -- 1320 MVar/LConn1 -- Load Flow Bus2/LConn1
  3800 MVA 17KV :650KV Transformer/LConn1 -- Load Flow Bus3/LConn1 -- MPP4-TEST2 96 km/LConn1
  "3700 MVA 17KV :650KV Transformer "/LConn2 -- 185 MW/LConn2 -- MPP1_3700MVA 17KV/RConn2
  MPP3-TEST2 111 km/RConn3 -- 660 MVar4/LConn1 -- MPP4-TEST2 96 km/RConn3 -- TEST2/LConn3
  TEST1-MPP2 187 km/RConn1 -- TEST 1/LConn3 -- TEST1-PNS 235 km/LConn3
  TEST2/RConn3 -- CLP-TEST2 288 km/LConn3
  MPP3-TEST2 111 km/RConn1 -- 660 MVar4/LConn3 -- MPP4-TEST2 96 km/RConn1 -- TEST2/LConn1
  Cs CLPS/LConn2 -- Cs AND/RConn2 -- CLP-TEST2 288 km/RConn2
  CLP-TEST2 288 km/RConn3 -- Cs CLPS/LConn3 -- Cs AND/RConn3
  800 MVA 17KV :650KV Transformer/LConn2 -- MPP3-TEST2 111 km/LConn2
  CSG 1/LConn3 -- Cs CSGN/RConn3
  MPP4_3800MVA 17KV/RConn2 -- 190 MW/LConn2 -- 3800 MVA 17KV :650KV Transformer/RConn2
  800 MVA 17KV :650KV Transformer/RConn2 -- 40 MW/LConn2 -- MPP3_800MVA 17KV/RConn2
  800 MVA 17KV :650KV Transformer/LConn1 -- MPP3-TEST2 111 km/LConn1
  MPP1-CLP 310 km/RConn1 -- Cs CLPN/LConn1
  MPP1-CLP 310 km/RConn3 -- Cs CLPN/LConn3
  TEST1-MPP2 187 km/LConn2 -- 1980 MVar/LConn2 -- "500 MVA 17KV :650KV Transformer "/LConn2
  TEST2/RConn1 -- Load Flow Bus5/LConn1 -- CLP-TEST2 288 km/LConn1
  MPP2_500MVA 17KV/RConn1 -- Load Flow Bus1/LConn1 -- 25 MW/LConn1 -- "500 MVA 17KV :650KV Transformer "/RConn1
  800 MVA 17KV :650KV Transformer/LConn3 -- MPP3-TEST2 111 km/LConn3
  MPP1-CLP 310 km/RConn2 -- Cs CLPN/LConn2
  CLP-CSG 103 km/RConn2 -- 990 MVar3/LConn2 -- CLP 1/RConn2
  CSG 1/LConn2 -- Cs CSGN/RConn2
  MPP3_800MVA 17KV/RConn3 -- 40 MW/LConn3 -- 800 MVA 17KV :650KV Transformer/RConn3
  CSG 1/LConn1 -- Cs CSGN/RConn1
  TEST2/RConn2 -- CLP-TEST2 288 km/LConn2
  3800 MVA 17KV :650KV Transformer/LConn3 -- MPP4-TEST2 96 km/LConn3
  Cs CSGN/LConn1 -- CLP-CSG 103 km/LConn1
  MPP5_4200MVA 17KV/RConn1 -- 210 MW/LConn1 -- 4200 MVA 17KV :650KV Transformer/LConn1 -- Load Flow Bus10/LConn1
  MPP5_4200MVA 17KV/RConn2 -- 210 MW/LConn2 -- 4200 MVA 17KV :650KV Transformer/LConn2
  MPP5_4200MVA 17KV/RConn3 -- 210 MW/LConn3 -- 4200 MVA 17KV :650KV Transformer/LConn3
  MPP6_490MVA 17KV/RConn1 -- 25 MW1/LConn1 -- 490 MVA 17KV :650KV Transformer/LConn1 -- Load Flow Bus12/LConn1
  MPP6_490MVA 17KV/RConn2 -- 25 MW1/LConn2 -- 490 MVA 17KV :650KV Transformer/LConn2
  MPP6_490MVA 17KV/RConn3 -- 25 MW1/LConn3 -- 490 MVA 17KV :650KV Transformer/LConn3
  Cs PNSM/LConn3 -- PNS3/RConn3
  Cs PNSM/LConn1 -- PNS3/RConn1
  Cs PNSM/LConn2 -- PNS3/RConn2
  Cs PNSN/RConn2 -- PNS3/LConn2
  PNS3/LConn3 -- Cs PNSN/RConn3
  Cs PNSN/RConn1 -- PNS3/LConn1 -- Load Flow Bus8/LConn1
  490 MVA 17KV :650KV Transformer/RConn1 -- 2310 MVar/LConn1 -- MPP6-CSG 186 km/LConn1
  490 MVA 17KV :650KV Transformer/RConn2 -- 2310 MVar/LConn2 -- MPP6-CSG 186 km/LConn2
  MPP6-CSG 186 km/RConn1 -- CSG 1/RConn1
  MPP6-CSG 186 km/RConn2 -- CSG 1/RConn2
  MPP6-CSG 186 km/RConn3 -- CSG 1/RConn3
  490 MVA 17KV :650KV Transformer/RConn3 -- 2310 MVar/LConn3 -- MPP6-CSG 186 km/LConn3
  SAT-a/RConn1 -- 660 MVar/LConn1 -- Cs SATS/RConn1
  SAT-b/RConn1 -- 660 MVar/LConn2 -- Cs SATS/RConn2
  SAT-c/RConn1 -- 660 MVar/LConn3 -- Cs SATS/RConn3
  Cs SATS/LConn3 -- " SAT-AND 129 km"/LConn3
  " SAT-AND 129 km"/LConn1 -- Cs SATS/LConn1
  Cs SATS/LConn2 -- " SAT-AND 129 km"/LConn2
  Cs PNSM/RConn1 -- TEST1-PNS 235 km/RConn1
  TEST1-PNS 235 km/RConn2 -- Cs PNSM/RConn2
  Cs PNSM/RConn3 -- TEST1-PNS 235 km/RConn3
  PNS-CON 260 km/LConn1 -- 990 MVar/LConn1 -- Cs PNSN/LConn1
  PNS-CON 260 km/LConn2 -- 990 MVar/LConn2 -- Cs PNSN/LConn2
  PNS-CON 260 km/LConn3 -- 990 MVar/LConn3 -- Cs PNSN/LConn3
  CON-a/RConn1 -- PNS-CON 260 km/RConn1
  CON-b/RConn1 -- PNS-CON 260 km/RConn2
  CON-c/RConn1 -- PNS-CON 260 km/RConn3
  AND1/RConn3 -- " SAT-AND 129 km"/RConn3
  AND1/RConn2 -- " SAT-AND 129 km"/RConn2
  AND1/RConn1 -- " SAT-AND 129 km"/RConn1
  Cs AND/LConn1 -- AND1/LConn1
  Cs AND/LConn3 -- Load Flow Bus11/LConn1 -- AND1/LConn3
  Cs AND/LConn2 -- AND1/LConn2
  TEST1-PNS 235 km/LConn1 -- TEST 1/LConn1 -- TEST1-MPP2 187 km/RConn3
  "3700 MVA 17KV :650KV Transformer "/RConn2 -- Cs MPP1D/RConn2 -- 1320 MVar/LConn2 -- MPP1-CLP 310 km/LConn2
  MPP1-CLP 310 km/LConn3 -- Cs MPP1D/RConn3 -- 1320 MVar/LConn3 -- "3700 MVA 17KV :650KV Transformer "/RConn3
  TEST 1/RConn1 -- Cs MPP1D/LConn1
  TEST 1/RConn2 -- Cs MPP1D/LConn2
  TEST 1/RConn3 -- Cs MPP1D/LConn3
